simulink model "myo_sfun_one_myo_imu_emg"  (R2019a)
(part 5 of 12)

  "IW{2,1}(261,:)'" : Constant  Value=[-0.5347940637473553859848607316962443292140960693359375;-0.259539238988193254886738259301637299358844757080078125;-0.7408074576731140670204922571429051458835601806640625;-0.40336307327878595518910742612206377089023590087890625;-1.55843068978388021861292145331390202045440673828125;1.7382673124555321209072644705884158611297607421875;1.5250036038475383026735698877018876373767852783203125;1.420255341369331514300711205578409135341644287109375]
      mask Display: e = 0.06;c1 = [120 150 230]/255;c2 = ([120 150 230]+0)/383;c3 = ([120 150 230]+128)/383;patch([0 1 1 0],[0 0 1 1],c1);patch([0 1 1 1-e 1-e 0+e],[0 0 1 1-e 0+e 0+e],c2);patch([0 0 1 1-e 0+e 0+e],[0 1 1 1-e 1-e 0+e],c3);plot([0 1 1 0 0],[0 0 1 1 0]);disp('weights');
  "IW{2,1}(262,:)'" : Constant  Value=[-1.2137447248221431284065374711644835770130157470703125;1.3683347708584874258264107993454672396183013916015625;1.5705948868795653883267959827207960188388824462890625;0.11601457680919935455676750279963016510009765625;0.762641288467723388322383470949716866016387939453125;0.40056359138445618572887951813754625618457794189453125;0.9697544812676659464756312445388175547122955322265625;-1.8867637485871338043352807289920747280120849609375]
      mask Display: e = 0.06;c1 = [120 150 230]/255;c2 = ([120 150 230]+0)/383;c3 = ([120 150 230]+128)/383;patch([0 1 1 0],[0 0 1 1],c1);patch([0 1 1 1-e 1-e 0+e],[0 0 1 1-e 0+e 0+e],c2);patch([0 0 1 1-e 0+e 0+e],[0 1 1 1-e 1-e 0+e],c3);plot([0 1 1 0 0],[0 0 1 1 0]);disp('weights');
  "IW{2,1}(263,:)'" : Constant  Value=[0.96222248705589408235283599424292333424091339111328125;-1.7544566772263916476504164165817201137542724609375;-0.7898635199195138678618377525708638131618499755859375;1.1345806161849127935425940449931658804416656494140625;1.2407133822809399692488341315765865147113800048828125;1.6768418735501995353587290082941763103008270263671875;0.8817648711825756269178100410499610006809234619140625;-0.3888922972442336867260337385232560336589813232421875]
      mask Display: e = 0.06;c1 = [120 150 230]/255;c2 = ([120 150 230]+0)/383;c3 = ([120 150 230]+128)/383;patch([0 1 1 0],[0 0 1 1],c1);patch([0 1 1 1-e 1-e 0+e],[0 0 1 1-e 0+e 0+e],c2);patch([0 0 1 1-e 0+e 0+e],[0 1 1 1-e 1-e 0+e],c3);plot([0 1 1 0 0],[0 0 1 1 0]);disp('weights');
  "IW{2,1}(264,:)'" : Constant  Value=[-1.5476465341889766857974564118194393813610076904296875;1.326692801950664080123942767386324703693389892578125;-1.4681341462454096102874245843850076198577880859375;-0.46925473122198557707207555722561664879322052001953125;1.2734078675367908051185850126785226166248321533203125;0.56485698316167909371898758763563819229602813720703125;-0.88411430126475953894527037846273742616176605224609375;1.345718049246266811991290524019859731197357177734375]
      mask Display: e = 0.06;c1 = [120 150 230]/255;c2 = ([120 150 230]+0)/383;c3 = ([120 150 230]+128)/383;patch([0 1 1 0],[0 0 1 1],c1);patch([0 1 1 1-e 1-e 0+e],[0 0 1 1-e 0+e 0+e],c2);patch([0 0 1 1-e 0+e 0+e],[0 1 1 1-e 1-e 0+e],c3);plot([0 1 1 0 0],[0 0 1 1 0]);disp('weights');
  "IW{2,1}(265,:)'" : Constant  Value=[1.3669130157252069590612109095673076808452606201171875;0.38000314021766767869081604658276773989200592041015625;1.4510424437195197366889942713896743953227996826171875;1.132229379854207795830234317691065371036529541015625;-0.7653685535385428284627096218173392117023468017578125;-1.6459644702436435625969579632510431110858917236328125;-1.210523284810293365154620914836414158344268798828125;-0.87108616897754220786964651779271662235260009765625]
      mask Display: e = 0.06;c1 = [120 150 230]/255;c2 = ([120 150 230]+0)/383;c3 = ([120 150 230]+128)/383;patch([0 1 1 0],[0 0 1 1],c1);patch([0 1 1 1-e 1-e 0+e],[0 0 1 1-e 0+e 0+e],c2);patch([0 0 1 1-e 0+e 0+e],[0 1 1 1-e 1-e 0+e],c3);plot([0 1 1 0 0],[0 0 1 1 0]);disp('weights');
  "IW{2,1}(266,:)'" : Constant  Value=[1.5789125748257089032478006629389710724353790283203125;-1.7464317776296429673976717822370119392871856689453125;0.989813563582735422841096806223504245281219482421875;0.93718327672771994940603690338321030139923095703125;-1.0300358206486419643255203482112847268581390380859375;-0.33243528081857032230317372523131780326366424560546875;-0.048545225170301485595469870304441428743302822113037109375;1.6203864687595086468974159288336522877216339111328125]
      mask Display: e = 0.06;c1 = [120 150 230]/255;c2 = ([120 150 230]+0)/383;c3 = ([120 150 230]+128)/383;patch([0 1 1 0],[0 0 1 1],c1);patch([0 1 1 1-e 1-e 0+e],[0 0 1 1-e 0+e 0+e],c2);patch([0 0 1 1-e 0+e 0+e],[0 1 1 1-e 1-e 0+e],c3);plot([0 1 1 0 0],[0 0 1 1 0]);disp('weights');
  "IW{2,1}(267,:)'" : Constant  Value=[-1.88334330389469162270188462571240961551666259765625;-1.550976382192118752101350764860399067401885986328125;1.4240772823814003000819639055407606065273284912109375;0.82226012569760731363288641659892164170742034912109375;-0.78530498389310732232360123816761188209056854248046875;-0.9885174017696252146691904272302053868770599365234375;0.9423763715994548650911610820912756025791168212890625;-0.4230164293665026331581202612142078578472137451171875]
      mask Display: e = 0.06;c1 = [120 150 230]/255;c2 = ([120 150 230]+0)/383;c3 = ([120 150 230]+128)/383;patch([0 1 1 0],[0 0 1 1],c1);patch([0 1 1 1-e 1-e 0+e],[0 0 1 1-e 0+e 0+e],c2);patch([0 0 1 1-e 0+e 0+e],[0 1 1 1-e 1-e 0+e],c3);plot([0 1 1 0 0],[0 0 1 1 0]);disp('weights');
  "IW{2,1}(268,:)'" : Constant  Value=[0.77703759880490519407203464652411639690399169921875;0.431370173463836492633305397248477675020694732666015625;-1.1019623341089503920642300727195106446743011474609375;1.719390729815739593533407969516701996326446533203125;0.70250763369316004958164967320044524967670440673828125;-1.8212153285883927456012543188990093767642974853515625;0.078282166399910979581733272425481118261814117431640625;1.5732714658743549573927111850935034453868865966796875]
      mask Display: e = 0.06;c1 = [120 150 230]/255;c2 = ([120 150 230]+0)/383;c3 = ([120 150 230]+128)/383;patch([0 1 1 0],[0 0 1 1],c1);patch([0 1 1 1-e 1-e 0+e],[0 0 1 1-e 0+e 0+e],c2);patch([0 0 1 1-e 0+e 0+e],[0 1 1 1-e 1-e 0+e],c3);plot([0 1 1 0 0],[0 0 1 1 0]);disp('weights');
  "IW{2,1}(269,:)'" : Constant  Value=[0.358805185099290657735338072598096914589405059814453125;-0.85788688273212521107069505887920968234539031982421875;0.6189663674455470054880379393580369651317596435546875;0.3732430252180132246309085530810989439487457275390625;-1.52643420461756118555740613373927772045135498046875;-0.8164779329250595463207673674332909286022186279296875;-1.966212472493690910368968616239726543426513671875;1.6658060255045030739751155124395154416561126708984375]
      mask Display: e = 0.06;c1 = [120 150 230]/255;c2 = ([120 150 230]+0)/383;c3 = ([120 150 230]+128)/383;patch([0 1 1 0],[0 0 1 1],c1);patch([0 1 1 1-e 1-e 0+e],[0 0 1 1-e 0+e 0+e],c2);patch([0 0 1 1-e 0+e 0+e],[0 1 1 1-e 1-e 0+e],c3);plot([0 1 1 0 0],[0 0 1 1 0]);disp('weights');
  "IW{2,1}(27,:)'" : Constant  Value=[1.0976471878022999728585773482336662709712982177734375;-1.466978524772944769694049682584591209888458251953125;-0.06567386280703979561934602315886877477169036865234375;-0.90721269995288233989327864037477411329746246337890625;-0.5755879150808522748405948732397519052028656005859375;-1.2134225702139129765555480844341218471527099609375;1.689553489070515723824428278021514415740966796875;-1.478611033845023126076512198778800666332244873046875]
      mask Display: e = 0.06;c1 = [120 150 230]/255;c2 = ([120 150 230]+0)/383;c3 = ([120 150 230]+128)/383;patch([0 1 1 0],[0 0 1 1],c1);patch([0 1 1 1-e 1-e 0+e],[0 0 1 1-e 0+e 0+e],c2);patch([0 0 1 1-e 0+e 0+e],[0 1 1 1-e 1-e 0+e],c3);plot([0 1 1 0 0],[0 0 1 1 0]);disp('weights');
  "IW{2,1}(270,:)'" : Constant  Value=[1.4595164985252182532349252142012119293212890625;-0.359501600059089099215015039590070955455303192138671875;0.096861650405547894404634234888362698256969451904296875;-1.49178391212668426391019238508306443691253662109375;1.389601437905864766975128077319823205471038818359375;0.373202055967952806003751220487174578011035919189453125;1.851491441376186042333529258030466735363006591796875;-1.073163490086033622361583184101618826389312744140625]
      mask Display: e = 0.06;c1 = [120 150 230]/255;c2 = ([120 150 230]+0)/383;c3 = ([120 150 230]+128)/383;patch([0 1 1 0],[0 0 1 1],c1);patch([0 1 1 1-e 1-e 0+e],[0 0 1 1-e 0+e 0+e],c2);patch([0 0 1 1-e 0+e 0+e],[0 1 1 1-e 1-e 0+e],c3);plot([0 1 1 0 0],[0 0 1 1 0]);disp('weights');
  "IW{2,1}(271,:)'" : Constant  Value=[0.97058856146866234748671331544755958020687103271484375;-0.65670569787586685617242210355470888316631317138671875;-0.5609898191570097392144589321105740964412689208984375;-0.9346593350875387340437328020925633609294891357421875;-0.9836655602936890119281088118441402912139892578125;2.248750882651939786427419676329009234905242919921875;-1.32453501057655298467352622537873685359954833984375;0.86687601885010667768227676788228563964366912841796875]
      mask Display: e = 0.06;c1 = [120 150 230]/255;c2 = ([120 150 230]+0)/383;c3 = ([120 150 230]+128)/383;patch([0 1 1 0],[0 0 1 1],c1);patch([0 1 1 1-e 1-e 0+e],[0 0 1 1-e 0+e 0+e],c2);patch([0 0 1 1-e 0+e 0+e],[0 1 1 1-e 1-e 0+e],c3);plot([0 1 1 0 0],[0 0 1 1 0]);disp('weights');
  "IW{2,1}(272,:)'" : Constant  Value=[-1.32787760878514671247785372543148696422576904296875;0.84357176605215411502314282188308425247669219970703125;0.455621916527780113082002344526699744164943695068359375;-0.7202920248291266869244964254903607070446014404296875;1.0883011856233171243957258411683142185211181640625;-1.6432271653339125538906273504835553467273712158203125;0.82982796555327198451124104394693858921527862548828125;1.7873354043180602612750362823135219514369964599609375]
      mask Display: e = 0.06;c1 = [120 150 230]/255;c2 = ([120 150 230]+0)/383;c3 = ([120 150 230]+128)/383;patch([0 1 1 0],[0 0 1 1],c1);patch([0 1 1 1-e 1-e 0+e],[0 0 1 1-e 0+e 0+e],c2);patch([0 0 1 1-e 0+e 0+e],[0 1 1 1-e 1-e 0+e],c3);plot([0 1 1 0 0],[0 0 1 1 0]);disp('weights');
  "IW{2,1}(273,:)'" : Constant  Value=[-1.43578424813973182239124071202240884304046630859375;-1.8517703535549074889132725729723460972309112548828125;0.41544081412662092755994081016979180276393890380859375;-1.091247752457320530083961784839630126953125;-0.196299549298969033817030549471382983028888702392578125;-0.95868845801884028379191704516415484249591827392578125;1.2310815496712879113516692086705006659030914306640625;-1.3264965863304400972566554628429003059864044189453125]
      mask Display: e = 0.06;c1 = [120 150 230]/255;c2 = ([120 150 230]+0)/383;c3 = ([120 150 230]+128)/383;patch([0 1 1 0],[0 0 1 1],c1);patch([0 1 1 1-e 1-e 0+e],[0 0 1 1-e 0+e 0+e],c2);patch([0 0 1 1-e 0+e 0+e],[0 1 1 1-e 1-e 0+e],c3);plot([0 1 1 0 0],[0 0 1 1 0]);disp('weights');
  "IW{2,1}(274,:)'" : Constant  Value=[-0.95662628683772410465024904624442569911479949951171875;-1.0981679705156925930253919432288967072963714599609375;1.5430734491925364171294177140225656330585479736328125;-0.1038975800053978659764908343277056701481342315673828125;1.3390766380696075277256795743596740067005157470703125;0.9747187685846545601719981277710758149623870849609375;-0.63364061371546254175513013251475058495998382568359375;1.841906858781021671944699846790172159671783447265625]
      mask Display: e = 0.06;c1 = [120 150 230]/255;c2 = ([120 150 230]+0)/383;c3 = ([120 150 230]+128)/383;patch([0 1 1 0],[0 0 1 1],c1);patch([0 1 1 1-e 1-e 0+e],[0 0 1 1-e 0+e 0+e],c2);patch([0 0 1 1-e 0+e 0+e],[0 1 1 1-e 1-e 0+e],c3);plot([0 1 1 0 0],[0 0 1 1 0]);disp('weights');
  "IW{2,1}(275,:)'" : Constant  Value=[-0.34169892612024443945273333156364969909191131591796875;-0.89637397571807053697767742050928063690662384033203125;1.1176334887777461535307566009578295052051544189453125;2.103754722856508774242456638603471219539642333984375;1.3408946331418707398341894077020697295665740966796875;-1.33424973593796547532974727801047265529632568359375;0.59089858131655770279166972613893449306488037109375;-0.7138255704883051944165117674856446683406829833984375]
      mask Display: e = 0.06;c1 = [120 150 230]/255;c2 = ([120 150 230]+0)/383;c3 = ([120 150 230]+128)/383;patch([0 1 1 0],[0 0 1 1],c1);patch([0 1 1 1-e 1-e 0+e],[0 0 1 1-e 0+e 0+e],c2);patch([0 0 1 1-e 0+e 0+e],[0 1 1 1-e 1-e 0+e],c3);plot([0 1 1 0 0],[0 0 1 1 0]);disp('weights');
  "IW{2,1}(276,:)'" : Constant  Value=[-1.3416184792027767702649043712881393730640411376953125;1.4813472558584823701721688848920166492462158203125;1.449577220120267018188542351708747446537017822265625;1.97812474261925874685630333260633051395416259765625;0.161596659980792811683869558692094869911670684814453125;-0.644855468938165810044438330805860459804534912109375;0.511488114681550865014969531330280005931854248046875;0.54368784143616533111043054304900579154491424560546875]
      mask Display: e = 0.06;c1 = [120 150 230]/255;c2 = ([120 150 230]+0)/383;c3 = ([120 150 230]+128)/383;patch([0 1 1 0],[0 0 1 1],c1);patch([0 1 1 1-e 1-e 0+e],[0 0 1 1-e 0+e 0+e],c2);patch([0 0 1 1-e 0+e 0+e],[0 1 1 1-e 1-e 0+e],c3);plot([0 1 1 0 0],[0 0 1 1 0]);disp('weights');
  "IW{2,1}(277,:)'" : Constant  Value=[-1.735736727684186408993127770372666418552398681640625;1.4868573855134827876867120721726678311824798583984375;-1.5646534212947937891868832593900151550769805908203125;0.400031089853374488551907006694818846881389617919921875;-0.024142580804420908646701349198337993584573268890380859375;0.780105394974893950887917526415549218654632568359375;0.85181123327748242690660163134452886879444122314453125;1.3627409629516336053711711429059505462646484375]
      mask Display: e = 0.06;c1 = [120 150 230]/255;c2 = ([120 150 230]+0)/383;c3 = ([120 150 230]+128)/383;patch([0 1 1 0],[0 0 1 1],c1);patch([0 1 1 1-e 1-e 0+e],[0 0 1 1-e 0+e 0+e],c2);patch([0 0 1 1-e 0+e 0+e],[0 1 1 1-e 1-e 0+e],c3);plot([0 1 1 0 0],[0 0 1 1 0]);disp('weights');
  "IW{2,1}(278,:)'" : Constant  Value=[-1.56186260805010501684364498942159116268157958984375;-1.100006899394458059759926982223987579345703125;1.560648778966891025987706598243676126003265380859375;1.4873168322882188707723116749548353254795074462890625;0.46043106493486385399904747828259132802486419677734375;0.185967771515183122321701603141264058649539947509765625;1.4417075965386454416972128456109203398227691650390625;-0.53803330954568850952313141533522866666316986083984375]
      mask Display: e = 0.06;c1 = [120 150 230]/255;c2 = ([120 150 230]+0)/383;c3 = ([120 150 230]+128)/383;patch([0 1 1 0],[0 0 1 1],c1);patch([0 1 1 1-e 1-e 0+e],[0 0 1 1-e 0+e 0+e],c2);patch([0 0 1 1-e 0+e 0+e],[0 1 1 1-e 1-e 0+e],c3);plot([0 1 1 0 0],[0 0 1 1 0]);disp('weights');
  "IW{2,1}(279,:)'" : Constant  Value=[-0.36281345583298441059838523869984783232212066650390625;1.4390043629114261936052798773744143545627593994140625;0.06453072679456033078349008746954496018588542938232421875;1.05104162461502159686688173678703606128692626953125;-1.5431302947782772339024859320488758385181427001953125;-0.93221088137758789660125557929859496653079986572265625;0.267812486808182315112247806609957478940486907958984375;2.097864843359056319371802601381205022335052490234375]
      mask Display: e = 0.06;c1 = [120 150 230]/255;c2 = ([120 150 230]+0)/383;c3 = ([120 150 230]+128)/383;patch([0 1 1 0],[0 0 1 1],c1);patch([0 1 1 1-e 1-e 0+e],[0 0 1 1-e 0+e 0+e],c2);patch([0 0 1 1-e 0+e 0+e],[0 1 1 1-e 1-e 0+e],c3);plot([0 1 1 0 0],[0 0 1 1 0]);disp('weights');
  "IW{2,1}(28,:)'" : Constant  Value=[-0.90251119652570188645057669418747536838054656982421875;1.9962297316221044862771805128431878983974456787109375;2.10309210297034088199552570586092770099639892578125;-1.0280337214971939641117160135763697326183319091796875;0.519169850362849683023114266688935458660125732421875;0.58015023794351805452862436141003854572772979736328125;0.1759229481877064016348555242075235582888126373291015625;0.326899828584390539365500671920017339289188385009765625]
      mask Display: e = 0.06;c1 = [120 150 230]/255;c2 = ([120 150 230]+0)/383;c3 = ([120 150 230]+128)/383;patch([0 1 1 0],[0 0 1 1],c1);patch([0 1 1 1-e 1-e 0+e],[0 0 1 1-e 0+e 0+e],c2);patch([0 0 1 1-e 0+e 0+e],[0 1 1 1-e 1-e 0+e],c3);plot([0 1 1 0 0],[0 0 1 1 0]);disp('weights');
  "IW{2,1}(280,:)'" : Constant  Value=[1.126874992238202199956731419661082327365875244140625;-0.310662957071799805675027528195641934871673583984375;1.3794381468792427103409181654569692909717559814453125;-1.1011192837083199069780903300852514803409576416015625;1.2389242018177260007405493524856865406036376953125;0.2294867389644391353353825024896650575101375579833984375;1.0441557628103759203241907016490586102008819580078125;1.9669664675496492112216628811438567936420440673828125]
      mask Display: e = 0.06;c1 = [120 150 230]/255;c2 = ([120 150 230]+0)/383;c3 = ([120 150 230]+128)/383;patch([0 1 1 0],[0 0 1 1],c1);patch([0 1 1 1-e 1-e 0+e],[0 0 1 1-e 0+e 0+e],c2);patch([0 0 1 1-e 0+e 0+e],[0 1 1 1-e 1-e 0+e],c3);plot([0 1 1 0 0],[0 0 1 1 0]);disp('weights');
  "IW{2,1}(281,:)'" : Constant  Value=[0.483592536764545333216602784887072630226612091064453125;-2.158889894419294019911603754735551774501800537109375;-1.05987617340272688437607939704321324825286865234375;0.69486367072161192570689536296413280069828033447265625;1.1198683344627422542316708131693303585052490234375;-1.1965790950295855932239419416873715817928314208984375;-0.9931210388714486470007614116184413433074951171875;-0.942888086306401529412823947495780885219573974609375]
      mask Display: e = 0.06;c1 = [120 150 230]/255;c2 = ([120 150 230]+0)/383;c3 = ([120 150 230]+128)/383;patch([0 1 1 0],[0 0 1 1],c1);patch([0 1 1 1-e 1-e 0+e],[0 0 1 1-e 0+e 0+e],c2);patch([0 0 1 1-e 0+e 0+e],[0 1 1 1-e 1-e 0+e],c3);plot([0 1 1 0 0],[0 0 1 1 0]);disp('weights');
  "IW{2,1}(282,:)'" : Constant  Value=[0.91468655581167979118362154622445814311504364013671875;-1.1775706258562699257907979699666611850261688232421875;-0.96927585702251750632285620667971670627593994140625;-1.3837978877602832294968493442866019904613494873046875;1.3407367494679702790705277948291040956974029541015625;1.075182371223083688249744227505289018154144287109375;-1.410665767931468916884796271915547549724578857421875;1.0674170493635213308181164393317885696887969970703125]
      mask Display: e = 0.06;c1 = [120 150 230]/255;c2 = ([120 150 230]+0)/383;c3 = ([120 150 230]+128)/383;patch([0 1 1 0],[0 0 1 1],c1);patch([0 1 1 1-e 1-e 0+e],[0 0 1 1-e 0+e 0+e],c2);patch([0 0 1 1-e 0+e 0+e],[0 1 1 1-e 1-e 0+e],c3);plot([0 1 1 0 0],[0 0 1 1 0]);disp('weights');
  "IW{2,1}(283,:)'" : Constant  Value=[-1.3783752363382208994124766832101158797740936279296875;1.0054603651816405029961742911837063729763031005859375;-1.494867039260532326494512744829989969730377197265625;1.0665452392347567478481096259201876819133758544921875;1.018899772728071528860027683549560606479644775390625;-1.285845475365987145011104075820185244083404541015625;-1.429423307222606798205788436462171375751495361328125;-0.10322951687595514902451299121821648441255092620849609375]
      mask Display: e = 0.06;c1 = [120 150 230]/255;c2 = ([120 150 230]+0)/383;c3 = ([120 150 230]+128)/383;patch([0 1 1 0],[0 0 1 1],c1);patch([0 1 1 1-e 1-e 0+e],[0 0 1 1-e 0+e 0+e],c2);patch([0 0 1 1-e 0+e 0+e],[0 1 1 1-e 1-e 0+e],c3);plot([0 1 1 0 0],[0 0 1 1 0]);disp('weights');
  "IW{2,1}(284,:)'" : Constant  Value=[0.1572972901949951374245273427732172422111034393310546875;-1.2723462678150279092648133882903493940830230712890625;1.561837886277977371918268545414321124553680419921875;1.741138590659697005236239419900812208652496337890625;0.83441033896946625869617264470434747636318206787109375;-0.039011284281160678311106693172405357472598552703857421875;1.7881067609712910648767092425259761512279510498046875;-0.2145482555579586725347240871997200883924961090087890625]
      mask Display: e = 0.06;c1 = [120 150 230]/255;c2 = ([120 150 230]+0)/383;c3 = ([120 150 230]+128)/383;patch([0 1 1 0],[0 0 1 1],c1);patch([0 1 1 1-e 1-e 0+e],[0 0 1 1-e 0+e 0+e],c2);patch([0 0 1 1-e 0+e 0+e],[0 1 1 1-e 1-e 0+e],c3);plot([0 1 1 0 0],[0 0 1 1 0]);disp('weights');
  "IW{2,1}(285,:)'" : Constant  Value=[-1.116838898596282714237304389826022088527679443359375;-0.45361005852011071493024019218864850699901580810546875;-0.1467195540551750887470205952922697179019451141357421875;-0.77123417068573274502085723725031130015850067138671875;-1.01269951209783659606955552590079605579376220703125;-1.536443689826322067659702952369116246700286865234375;0.7644814837354527714552432371419854462146759033203125;2.219712582372310283318483925540931522846221923828125]
      mask Display: e = 0.06;c1 = [120 150 230]/255;c2 = ([120 150 230]+0)/383;c3 = ([120 150 230]+128)/383;patch([0 1 1 0],[0 0 1 1],c1);patch([0 1 1 1-e 1-e 0+e],[0 0 1 1-e 0+e 0+e],c2);patch([0 0 1 1-e 0+e 0+e],[0 1 1 1-e 1-e 0+e],c3);plot([0 1 1 0 0],[0 0 1 1 0]);disp('weights');
  "IW{2,1}(286,:)'" : Constant  Value=[0.1995306126975101845832938352032215334475040435791015625;-1.7161681488379654236808846690109930932521820068359375;-1.480581408540153187658461320097558200359344482421875;-1.537504376924896387635044447961263358592987060546875;-1.7887266527028222729001072366372682154178619384765625;-0.1609063893290709479355626854157890193164348602294921875;0.05322388997146536293580965093497070483863353729248046875;-0.50484691917346913303532573991105891764163970947265625]
      mask Display: e = 0.06;c1 = [120 150 230]/255;c2 = ([120 150 230]+0)/383;c3 = ([120 150 230]+128)/383;patch([0 1 1 0],[0 0 1 1],c1);patch([0 1 1 1-e 1-e 0+e],[0 0 1 1-e 0+e 0+e],c2);patch([0 0 1 1-e 0+e 0+e],[0 1 1 1-e 1-e 0+e],c3);plot([0 1 1 0 0],[0 0 1 1 0]);disp('weights');
  "IW{2,1}(287,:)'" : Constant  Value=[-0.94112595153402944792020434761070646345615386962890625;-0.99001731697002182119859980957699008285999298095703125;1.8620901433696148696839145486592315137386322021484375;-0.6551074243207744007833071009372361004352569580078125;-0.1610648165904539907966608325295965187251567840576171875;0.89392555591680811222232705404167063534259796142578125;-2.086354445914893052105298920650966465473175048828125;-0.1826483784180093772331332502290024422109127044677734375]
      mask Display: e = 0.06;c1 = [120 150 230]/255;c2 = ([120 150 230]+0)/383;c3 = ([120 150 230]+128)/383;patch([0 1 1 0],[0 0 1 1],c1);patch([0 1 1 1-e 1-e 0+e],[0 0 1 1-e 0+e 0+e],c2);patch([0 0 1 1-e 0+e 0+e],[0 1 1 1-e 1-e 0+e],c3);plot([0 1 1 0 0],[0 0 1 1 0]);disp('weights');
  "IW{2,1}(288,:)'" : Constant  Value=[0.52458174714693217577377026827889494597911834716796875;1.7398230354122528051874496668460778892040252685546875;-1.519901214688633928062699851579964160919189453125;-0.86917209525089400568020892023923806846141815185546875;0.92940725891443654038681643214658834040164947509765625;1.2385217255743719011462644630228169262409210205078125;-1.58607583101517501944499599630944430828094482421875;-0.1160806490231749144026451858735526911914348602294921875]
      mask Display: e = 0.06;c1 = [120 150 230]/255;c2 = ([120 150 230]+0)/383;c3 = ([120 150 230]+128)/383;patch([0 1 1 0],[0 0 1 1],c1);patch([0 1 1 1-e 1-e 0+e],[0 0 1 1-e 0+e 0+e],c2);patch([0 0 1 1-e 0+e 0+e],[0 1 1 1-e 1-e 0+e],c3);plot([0 1 1 0 0],[0 0 1 1 0]);disp('weights');
  "IW{2,1}(289,:)'" : Constant  Value=[-1.2917048065390790423379030471551232039928436279296875;-0.71049630680784592318133263688650913536548614501953125;0.86402303793719081870250420251977629959583282470703125;-1.1367972813391349351519465926685370504856109619140625;1.765463373969804905527780647389590740203857421875;-0.39553717415411515645473627955652773380279541015625;-1.3503491957773159359845749349915422499179840087890625;1.303257147695879414328601342276670038700103759765625]
      mask Display: e = 0.06;c1 = [120 150 230]/255;c2 = ([120 150 230]+0)/383;c3 = ([120 150 230]+128)/383;patch([0 1 1 0],[0 0 1 1],c1);patch([0 1 1 1-e 1-e 0+e],[0 0 1 1-e 0+e 0+e],c2);patch([0 0 1 1-e 0+e 0+e],[0 1 1 1-e 1-e 0+e],c3);plot([0 1 1 0 0],[0 0 1 1 0]);disp('weights');
  "IW{2,1}(29,:)'" : Constant  Value=[-1.7090129519907464317185485924710519611835479736328125;-1.3034815042726444200837931930436752736568450927734375;-1.351266315762916558895767593639902770519256591796875;0.67773782565702356261994054875685833394527435302734375;0.78014348610426365038250651195994578301906585693359375;-0.62637339626419696880788023918285034596920013427734375;-1.20017218462587482719072795589454472064971923828125;1.4139008249440487841042113359435461461544036865234375]
      mask Display: e = 0.06;c1 = [120 150 230]/255;c2 = ([120 150 230]+0)/383;c3 = ([120 150 230]+128)/383;patch([0 1 1 0],[0 0 1 1],c1);patch([0 1 1 1-e 1-e 0+e],[0 0 1 1-e 0+e 0+e],c2);patch([0 0 1 1-e 0+e 0+e],[0 1 1 1-e 1-e 0+e],c3);plot([0 1 1 0 0],[0 0 1 1 0]);disp('weights');
  "IW{2,1}(290,:)'" : Constant  Value=[0.56386891610408518271668754096026532351970672607421875;-0.08552175739171119506210061445017345249652862548828125;1.1462792767544254246558921295218169689178466796875;-1.68939509070532078993664981680922210216522216796875;1.6352454019301372323269561093184165656566619873046875;1.517885155302728161785807969863526523113250732421875;-0.56379379957213171525864936484140343964099884033203125;1.0920500642273209823684965158463455736637115478515625]
      mask Display: e = 0.06;c1 = [120 150 230]/255;c2 = ([120 150 230]+0)/383;c3 = ([120 150 230]+128)/383;patch([0 1 1 0],[0 0 1 1],c1);patch([0 1 1 1-e 1-e 0+e],[0 0 1 1-e 0+e 0+e],c2);patch([0 0 1 1-e 0+e 0+e],[0 1 1 1-e 1-e 0+e],c3);plot([0 1 1 0 0],[0 0 1 1 0]);disp('weights');
  "IW{2,1}(291,:)'" : Constant  Value=[1.23373218350272306764736640616320073604583740234375;-1.3373685199427944869654538706527091562747955322265625;0.48442904663986230406891309030470438301563262939453125;-0.1576922269796413866860262942282133735716342926025390625;0.417134833136712346313146326792775653302669525146484375;0.74684790145846158271325521127437241375446319580078125;-1.515155489828451162992450917954556643962860107421875;2.1078436254838255337062946637161076068878173828125]
      mask Display: e = 0.06;c1 = [120 150 230]/255;c2 = ([120 150 230]+0)/383;c3 = ([120 150 230]+128)/383;patch([0 1 1 0],[0 0 1 1],c1);patch([0 1 1 1-e 1-e 0+e],[0 0 1 1-e 0+e 0+e],c2);patch([0 0 1 1-e 0+e 0+e],[0 1 1 1-e 1-e 0+e],c3);plot([0 1 1 0 0],[0 0 1 1 0]);disp('weights');
  "IW{2,1}(292,:)'" : Constant  Value=[0.149355769972121577016110904878587462007999420166015625;-1.797772213812643737895768936141394078731536865234375;1.7712538370147437039037185968481935560703277587890625;-1.0021657351335420127469433282385580241680145263671875;0.1743328572903561635154545683690230362117290496826171875;-1.4389073129166494169339785003103315830230712890625;-0.87641589879673664764681007000035606324672698974609375;0.8661315996802823047318042881670407950878143310546875]
      mask Display: e = 0.06;c1 = [120 150 230]/255;c2 = ([120 150 230]+0)/383;c3 = ([120 150 230]+128)/383;patch([0 1 1 0],[0 0 1 1],c1);patch([0 1 1 1-e 1-e 0+e],[0 0 1 1-e 0+e 0+e],c2);patch([0 0 1 1-e 0+e 0+e],[0 1 1 1-e 1-e 0+e],c3);plot([0 1 1 0 0],[0 0 1 1 0]);disp('weights');
  "IW{2,1}(293,:)'" : Constant  Value=[0.15491241101211217223720950642018578946590423583984375;0.16704681014463995669672158328467048704624176025390625;-1.0391931780589243050627601405722089111804962158203125;-2.043870802913976714165755765861831605434417724609375;-1.8472817074879319676483646617271006107330322265625;1.2477502395181587768746567235211841762065887451171875;-0.88279567899519839624389305754448287189006805419921875;0.03624299588909961344906918156993924640119075775146484375]
      mask Display: e = 0.06;c1 = [120 150 230]/255;c2 = ([120 150 230]+0)/383;c3 = ([120 150 230]+128)/383;patch([0 1 1 0],[0 0 1 1],c1);patch([0 1 1 1-e 1-e 0+e],[0 0 1 1-e 0+e 0+e],c2);patch([0 0 1 1-e 0+e 0+e],[0 1 1 1-e 1-e 0+e],c3);plot([0 1 1 0 0],[0 0 1 1 0]);disp('weights');
  "IW{2,1}(294,:)'" : Constant  Value=[-1.5072503309985483266331129925674758851528167724609375;-0.5912296405544983368685052482760511338710784912109375;-1.8839554420834103698467743015498854219913482666015625;-0.211657758410721930086850761654204688966274261474609375;-0.287930466127750139815333341175573877990245819091796875;0.281307788952104342872218012416851706802845001220703125;-1.9679232919960212289112178041250444948673248291015625;-0.80560222171074702401938338880427181720733642578125]
      mask Display: e = 0.06;c1 = [120 150 230]/255;c2 = ([120 150 230]+0)/383;c3 = ([120 150 230]+128)/383;patch([0 1 1 0],[0 0 1 1],c1);patch([0 1 1 1-e 1-e 0+e],[0 0 1 1-e 0+e 0+e],c2);patch([0 0 1 1-e 0+e 0+e],[0 1 1 1-e 1-e 0+e],c3);plot([0 1 1 0 0],[0 0 1 1 0]);disp('weights');
  "IW{2,1}(295,:)'" : Constant  Value=[0.12344705431950199481239138776800245977938175201416015625;-1.6339196595745466566995673929341137409210205078125;1.674123558913491738309176071197725832462310791015625;1.6729989118184416252432811234029941260814666748046875;0.54506681304176629598856607117340900003910064697265625;0.708510405456726832795766313211061060428619384765625;1.3533935295393735298574711123364977538585662841796875;-0.26785656899876630898660323509830050170421600341796875]
      mask Display: e = 0.06;c1 = [120 150 230]/255;c2 = ([120 150 230]+0)/383;c3 = ([120 150 230]+128)/383;patch([0 1 1 0],[0 0 1 1],c1);patch([0 1 1 1-e 1-e 0+e],[0 0 1 1-e 0+e 0+e],c2);patch([0 0 1 1-e 0+e 0+e],[0 1 1 1-e 1-e 0+e],c3);plot([0 1 1 0 0],[0 0 1 1 0]);disp('weights');
  "IW{2,1}(296,:)'" : Constant  Value=[-1.3048676985666547434306039576767943799495697021484375;1.643205394783701311922641252749599516391754150390625;0.1963040358895786763326896107173524796962738037109375;-1.244179839042650836944403636152856051921844482421875;0.930456184365194172158908259007148444652557373046875;-0.3428724376575236210129560276982374489307403564453125;-1.9619371156705327496894142313976772129535675048828125;-0.7667766256128121238333505971240811049938201904296875]
      mask Display: e = 0.06;c1 = [120 150 230]/255;c2 = ([120 150 230]+0)/383;c3 = ([120 150 230]+128)/383;patch([0 1 1 0],[0 0 1 1],c1);patch([0 1 1 1-e 1-e 0+e],[0 0 1 1-e 0+e 0+e],c2);patch([0 0 1 1-e 0+e 0+e],[0 1 1 1-e 1-e 0+e],c3);plot([0 1 1 0 0],[0 0 1 1 0]);disp('weights');
  "IW{2,1}(297,:)'" : Constant  Value=[0.7318966623372527013913213522755540907382965087890625;0.98989772384461360843488364480435848236083984375;-1.4657202518633074550535866364953108131885528564453125;-0.67854688032233922978520013202796690165996551513671875;-0.739015982277783312071051113889552652835845947265625;-1.4522550716225806066717041176161728799343109130859375;1.6168939132434669847526720332098193466663360595703125;-1.2758844453122988316096098060370422899723052978515625]
      mask Display: e = 0.06;c1 = [120 150 230]/255;c2 = ([120 150 230]+0)/383;c3 = ([120 150 230]+128)/383;patch([0 1 1 0],[0 0 1 1],c1);patch([0 1 1 1-e 1-e 0+e],[0 0 1 1-e 0+e 0+e],c2);patch([0 0 1 1-e 0+e 0+e],[0 1 1 1-e 1-e 0+e],c3);plot([0 1 1 0 0],[0 0 1 1 0]);disp('weights');
  "IW{2,1}(298,:)'" : Constant  Value=[1.209392504203771867565819775336422026157379150390625;1.2760262193505449435093623833381570875644683837890625;-0.66825151936986804113161042550927959382534027099609375;-1.694680276642486216331917603383772075176239013671875;-0.99422304321615195821237875861697830259799957275390625;-0.03750831860010338247857220039804815314710140228271484375;-1.392430533587185603749958318076096475124359130859375;-1.2927934329263728319148185619269497692584991455078125]
      mask Display: e = 0.06;c1 = [120 150 230]/255;c2 = ([120 150 230]+0)/383;c3 = ([120 150 230]+128)/383;patch([0 1 1 0],[0 0 1 1],c1);patch([0 1 1 1-e 1-e 0+e],[0 0 1 1-e 0+e 0+e],c2);patch([0 0 1 1-e 0+e 0+e],[0 1 1 1-e 1-e 0+e],c3);plot([0 1 1 0 0],[0 0 1 1 0]);disp('weights');
  "IW{2,1}(299,:)'" : Constant  Value=[0.7575431891216286572898752638138830661773681640625;1.229213305581662307730539396288804709911346435546875;1.810083283739304160775418495177291333675384521484375;-0.1572310105014219361319049994563101790845394134521484375;-0.89747854557077177961588176913210190832614898681640625;-1.1192368173888407323346427801880054175853729248046875;0.7573089087472901770325961479102261364459991455078125;-1.79694214217461034621692306245677173137664794921875]
      mask Display: e = 0.06;c1 = [120 150 230]/255;c2 = ([120 150 230]+0)/383;c3 = ([120 150 230]+128)/383;patch([0 1 1 0],[0 0 1 1],c1);patch([0 1 1 1-e 1-e 0+e],[0 0 1 1-e 0+e 0+e],c2);patch([0 0 1 1-e 0+e 0+e],[0 1 1 1-e 1-e 0+e],c3);plot([0 1 1 0 0],[0 0 1 1 0]);disp('weights');
  "IW{2,1}(3,:)'" : Constant  Value=[-0.83690372965789172621242641980643384158611297607421875;-1.154914680191724496438610003679059445858001708984375;1.13904575215728431913930762675590813159942626953125;0.95361878259994081741268701080116443336009979248046875;1.0615310460876534737195697744027711451053619384765625;0.286424987747621262457187185646034777164459228515625;-1.672805025225078789929966660565696656703948974609375;1.6609915496172871218760747069609351456165313720703125]
      mask Display: e = 0.06;c1 = [120 150 230]/255;c2 = ([120 150 230]+0)/383;c3 = ([120 150 230]+128)/383;patch([0 1 1 0],[0 0 1 1],c1);patch([0 1 1 1-e 1-e 0+e],[0 0 1 1-e 0+e 0+e],c2);patch([0 0 1 1-e 0+e 0+e],[0 1 1 1-e 1-e 0+e],c3);plot([0 1 1 0 0],[0 0 1 1 0]);disp('weights');
  "IW{2,1}(30,:)'" : Constant  Value=[-0.8706022673904982855930256846477277576923370361328125;-0.0879880741568741242542017744199256412684917449951171875;-0.323123551430262445638419421811704523861408233642578125;2.02198320106408768737082937150262296199798583984375;-0.86868500420774619197317178986850194633007049560546875;1.5624300902894974196755129014491103589534759521484375;1.6535207444727422210206668751197867095470428466796875;0.363206518091484298338400549255311489105224609375]
      mask Display: e = 0.06;c1 = [120 150 230]/255;c2 = ([120 150 230]+0)/383;c3 = ([120 150 230]+128)/383;patch([0 1 1 0],[0 0 1 1],c1);patch([0 1 1 1-e 1-e 0+e],[0 0 1 1-e 0+e 0+e],c2);patch([0 0 1 1-e 0+e 0+e],[0 1 1 1-e 1-e 0+e],c3);plot([0 1 1 0 0],[0 0 1 1 0]);disp('weights');
  "IW{2,1}(300,:)'" : Constant  Value=[-0.4695024464110899575786106652230955660343170166015625;-1.203705732039551445922143102507106959819793701171875;1.5130380234864684307893867298844270408153533935546875;1.3198736861827431443572322677937336266040802001953125;0.94438292148976887840916560890036635100841522216796875;-1.257930292994181353805061007733456790447235107421875;0.6973943764304555426036813514656387269496917724609375;1.5243184165398451224149312110967002809047698974609375]
      mask Display: e = 0.06;c1 = [120 150 230]/255;c2 = ([120 150 230]+0)/383;c3 = ([120 150 230]+128)/383;patch([0 1 1 0],[0 0 1 1],c1);patch([0 1 1 1-e 1-e 0+e],[0 0 1 1-e 0+e 0+e],c2);patch([0 0 1 1-e 0+e 0+e],[0 1 1 1-e 1-e 0+e],c3);plot([0 1 1 0 0],[0 0 1 1 0]);disp('weights');
  "IW{2,1}(301,:)'" : Constant  Value=[1.4992730582447182374750127564766444265842437744140625;-1.171026328408421246507487012422643601894378662109375;-0.5802693343082570009983101044781506061553955078125;-0.265006801952717252479629905792535282671451568603515625;0.8986575966217895672372151238960213959217071533203125;-1.120628035919562393019077717326581478118896484375;0.0262365055607453843966592188508002436719834804534912109375;-2.2217585154337573527527638361789286136627197265625]
      mask Display: e = 0.06;c1 = [120 150 230]/255;c2 = ([120 150 230]+0)/383;c3 = ([120 150 230]+128)/383;patch([0 1 1 0],[0 0 1 1],c1);patch([0 1 1 1-e 1-e 0+e],[0 0 1 1-e 0+e 0+e],c2);patch([0 0 1 1-e 0+e 0+e],[0 1 1 1-e 1-e 0+e],c3);plot([0 1 1 0 0],[0 0 1 1 0]);disp('weights');
  "IW{2,1}(302,:)'" : Constant  Value=[0.21645160550166575585961936667445115745067596435546875;1.7280621165898637503488544098217971622943878173828125;-1.115894301542621036560376523993909358978271484375;-0.99211020457547594020297765382565557956695556640625;-0.460189482165866914353813399429782293736934661865234375;1.2553463408558072078591294484795071184635162353515625;0.97984291896522612841380350801046006381511688232421875;-1.7219603540277537145897213122225366532802581787109375]
      mask Display: e = 0.06;c1 = [120 150 230]/255;c2 = ([120 150 230]+0)/383;c3 = ([120 150 230]+128)/383;patch([0 1 1 0],[0 0 1 1],c1);patch([0 1 1 1-e 1-e 0+e],[0 0 1 1-e 0+e 0+e],c2);patch([0 0 1 1-e 0+e 0+e],[0 1 1 1-e 1-e 0+e],c3);plot([0 1 1 0 0],[0 0 1 1 0]);disp('weights');
  "IW{2,1}(303,:)'" : Constant  Value=[-1.577092748516073061892939222161658108234405517578125;1.0490463847864577306978617343702353537082672119140625;0.2235141932496018946086024925534729845821857452392578125;-1.4370937545338706708974996217875741422176361083984375;-0.320615855533113391917510170969762839376926422119140625;-1.4147879504585691989859697059728205204010009765625;1.202651104290481054448491704533807933330535888671875;-1.3977749395487675254656778633943758904933929443359375]
      mask Display: e = 0.06;c1 = [120 150 230]/255;c2 = ([120 150 230]+0)/383;c3 = ([120 150 230]+128)/383;patch([0 1 1 0],[0 0 1 1],c1);patch([0 1 1 1-e 1-e 0+e],[0 0 1 1-e 0+e 0+e],c2);patch([0 0 1 1-e 0+e 0+e],[0 1 1 1-e 1-e 0+e],c3);plot([0 1 1 0 0],[0 0 1 1 0]);disp('weights');
  "IW{2,1}(304,:)'" : Constant  Value=[0.95787182259439707099346605900791473686695098876953125;1.2051911870966500739399407393648289144039154052734375;1.175954113818607371655389215447939932346343994140625;-0.80872558624624779621825609865481965243816375732421875;-1.9341362336565512958230783624458126723766326904296875;-0.7913495011414168889274378670961596071720123291015625;-0.58319732273415747503264583428972400724887847900390625;-1.405435564894582878281426019384525716304779052734375]
      mask Display: e = 0.06;c1 = [120 150 230]/255;c2 = ([120 150 230]+0)/383;c3 = ([120 150 230]+128)/383;patch([0 1 1 0],[0 0 1 1],c1);patch([0 1 1 1-e 1-e 0+e],[0 0 1 1-e 0+e 0+e],c2);patch([0 0 1 1-e 0+e 0+e],[0 1 1 1-e 1-e 0+e],c3);plot([0 1 1 0 0],[0 0 1 1 0]);disp('weights');
  "IW{2,1}(305,:)'" : Constant  Value=[0.0232546618312756796231877132186127710156142711639404296875;-1.6267041491998106561567283279146067798137664794921875;-0.68505978158889624385352590252296067774295806884765625;0.600360426501180821645675678155384957790374755859375;-1.644927790605635209431056864559650421142578125;0.29752486775745634606238354535889811813831329345703125;2.061487220312472334882158975233323872089385986328125;-0.74776707636719985661244436414563097059726715087890625]
      mask Display: e = 0.06;c1 = [120 150 230]/255;c2 = ([120 150 230]+0)/383;c3 = ([120 150 230]+128)/383;patch([0 1 1 0],[0 0 1 1],c1);patch([0 1 1 1-e 1-e 0+e],[0 0 1 1-e 0+e 0+e],c2);patch([0 0 1 1-e 0+e 0+e],[0 1 1 1-e 1-e 0+e],c3);plot([0 1 1 0 0],[0 0 1 1 0]);disp('weights');
  "IW{2,1}(306,:)'" : Constant  Value=[0.307643507114700398563655880934675224125385284423828125;-1.7516940236946150211139183738850988447666168212890625;-1.339174217498975139051253790967166423797607421875;-0.50228666573348423884937119510141201317310333251953125;1.658098944714120559495995621546171605587005615234375;-0.954504314461473324371354465256445109844207763671875;1.3790483009797374069904662974295206367969512939453125;-0.5206775011140762909889190268586389720439910888671875]
      mask Display: e = 0.06;c1 = [120 150 230]/255;c2 = ([120 150 230]+0)/383;c3 = ([120 150 230]+128)/383;patch([0 1 1 0],[0 0 1 1],c1);patch([0 1 1 1-e 1-e 0+e],[0 0 1 1-e 0+e 0+e],c2);patch([0 0 1 1-e 0+e 0+e],[0 1 1 1-e 1-e 0+e],c3);plot([0 1 1 0 0],[0 0 1 1 0]);disp('weights');
  "IW{2,1}(307,:)'" : Constant  Value=[-2.036521733314567317307819394045509397983551025390625;-1.0843540474509556492677120331791229546070098876953125;-0.978043574355647482576614493154920637607574462890625;1.20291024816412317477443139068782329559326171875;0.07484893373486158074658902705778018571436405181884765625;-0.9633395431981062184689790228730998933315277099609375;1.218326453460640390602520710672251880168914794921875;-0.9428558183991169183713054735562764108180999755859375]
      mask Display: e = 0.06;c1 = [120 150 230]/255;c2 = ([120 150 230]+0)/383;c3 = ([120 150 230]+128)/383;patch([0 1 1 0],[0 0 1 1],c1);patch([0 1 1 1-e 1-e 0+e],[0 0 1 1-e 0+e 0+e],c2);patch([0 0 1 1-e 0+e 0+e],[0 1 1 1-e 1-e 0+e],c3);plot([0 1 1 0 0],[0 0 1 1 0]);disp('weights');
  "IW{2,1}(308,:)'" : Constant  Value=[-0.343697267399743100479980739692109636962413787841796875;-2.357305464479904077990113364649005234241485595703125;0.82850372760230717172902359379804693162441253662109375;-0.6411439272598438154915356790297664701938629150390625;0.08881403549962600674216872675970080308616161346435546875;-0.5011156454033380835966227095923386514186859130859375;1.820618658772904741027787167695350944995880126953125;-0.67047534773334305224778972842614166438579559326171875]
      mask Display: e = 0.06;c1 = [120 150 230]/255;c2 = ([120 150 230]+0)/383;c3 = ([120 150 230]+128)/383;patch([0 1 1 0],[0 0 1 1],c1);patch([0 1 1 1-e 1-e 0+e],[0 0 1 1-e 0+e 0+e],c2);patch([0 0 1 1-e 0+e 0+e],[0 1 1 1-e 1-e 0+e],c3);plot([0 1 1 0 0],[0 0 1 1 0]);disp('weights');
  "IW{2,1}(309,:)'" : Constant  Value=[-1.818679086724649618389548777486197650432586669921875;-0.0225100328944918652573914386039177770726382732391357421875;-1.2850894056110899743572417719406075775623321533203125;0.58506139016945468700470200928975827991962432861328125;0.49690343152257998582399523002095520496368408203125;-2.300348438279462559563626200542785227298736572265625;0.274003116541775504355626935648615472018718719482421875;-0.282474236572137382683678197281551547348499298095703125]
      mask Display: e = 0.06;c1 = [120 150 230]/255;c2 = ([120 150 230]+0)/383;c3 = ([120 150 230]+128)/383;patch([0 1 1 0],[0 0 1 1],c1);patch([0 1 1 1-e 1-e 0+e],[0 0 1 1-e 0+e 0+e],c2);patch([0 0 1 1-e 0+e 0+e],[0 1 1 1-e 1-e 0+e],c3);plot([0 1 1 0 0],[0 0 1 1 0]);disp('weights');
  "IW{2,1}(31,:)'" : Constant  Value=[-0.6778220352334505260927244307822547852993011474609375;-1.002948065510846920034282447886653244495391845703125;0.01407924362783327144887923765281811938621103763580322265625;-1.65265069497485228566802106797695159912109375;-1.8678963103245307397770602619857527315616607666015625;1.6781190401603034434430128385429270565509796142578125;0.4976509515009865936008282005786895751953125;0.052912337285146604504149081549257971346378326416015625]
      mask Display: e = 0.06;c1 = [120 150 230]/255;c2 = ([120 150 230]+0)/383;c3 = ([120 150 230]+128)/383;patch([0 1 1 0],[0 0 1 1],c1);patch([0 1 1 1-e 1-e 0+e],[0 0 1 1-e 0+e 0+e],c2);patch([0 0 1 1-e 0+e 0+e],[0 1 1 1-e 1-e 0+e],c3);plot([0 1 1 0 0],[0 0 1 1 0]);disp('weights');
  "IW{2,1}(310,:)'" : Constant  Value=[-0.9850737716051496395408548778505064547061920166015625;1.0636727649987989252622355706989765167236328125;-1.282862670891714795828875139704905450344085693359375;1.4226035718425353859828419444966129958629608154296875;1.3300607573897007540608683484606444835662841796875;-0.312953405537495898958155748914577998220920562744140625;-1.392344087340662728280449300655163824558258056640625;-1.0806948454210629773086793647962622344493865966796875]
      mask Display: e = 0.06;c1 = [120 150 230]/255;c2 = ([120 150 230]+0)/383;c3 = ([120 150 230]+128)/383;patch([0 1 1 0],[0 0 1 1],c1);patch([0 1 1 1-e 1-e 0+e],[0 0 1 1-e 0+e 0+e],c2);patch([0 0 1 1-e 0+e 0+e],[0 1 1 1-e 1-e 0+e],c3);plot([0 1 1 0 0],[0 0 1 1 0]);disp('weights');
  "IW{2,1}(311,:)'" : Constant  Value=[-0.49294553067137314439349893291364423930644989013671875;-1.9141901169723762876628825324587523937225341796875;-0.778270681123441221416214830242097377777099609375;-0.509205764484566003602594719268381595611572265625;-1.5227342365238640820024329514126293361186981201171875;1.628009143875833064640801239875145256519317626953125;1.15603318056876336328286924981512129306793212890625;0.031259373196099560221483670829911716282367706298828125]
      mask Display: e = 0.06;c1 = [120 150 230]/255;c2 = ([120 150 230]+0)/383;c3 = ([120 150 230]+128)/383;patch([0 1 1 0],[0 0 1 1],c1);patch([0 1 1 1-e 1-e 0+e],[0 0 1 1-e 0+e 0+e],c2);patch([0 0 1 1-e 0+e 0+e],[0 1 1 1-e 1-e 0+e],c3);plot([0 1 1 0 0],[0 0 1 1 0]);disp('weights');
  "IW{2,1}(312,:)'" : Constant  Value=[-0.92467661683877022671396161968004889786243438720703125;-0.10371882087682215978219346652622334659099578857421875;0.2472184768976093127701432194953667931258678436279296875;-1.636317894696662111897467184462584555149078369140625;1.3811472962270487929714590791263617575168609619140625;-0.33054749103647285135565425662207417190074920654296875;2.0426896508592786716462796903215348720550537109375;-1.2247719007705752947146038422943092882633209228515625]
      mask Display: e = 0.06;c1 = [120 150 230]/255;c2 = ([120 150 230]+0)/383;c3 = ([120 150 230]+128)/383;patch([0 1 1 0],[0 0 1 1],c1);patch([0 1 1 1-e 1-e 0+e],[0 0 1 1-e 0+e 0+e],c2);patch([0 0 1 1-e 0+e 0+e],[0 1 1 1-e 1-e 0+e],c3);plot([0 1 1 0 0],[0 0 1 1 0]);disp('weights');
  "IW{2,1}(313,:)'" : Constant  Value=[-1.6957828522094453571611438746913336217403411865234375;-0.8732839118050577109642063078354112803936004638671875;-0.677899071672815267675105133093893527984619140625;0.04858513887136466091742903472550096921622753143310546875;1.6130422595957825127044316104729659855365753173828125;1.062862964497595985591260614455677568912506103515625;-1.743369601694128245839010560302995145320892333984375;0.048899058400884438946309984430627082474529743194580078125]
      mask Display: e = 0.06;c1 = [120 150 230]/255;c2 = ([120 150 230]+0)/383;c3 = ([120 150 230]+128)/383;patch([0 1 1 0],[0 0 1 1],c1);patch([0 1 1 1-e 1-e 0+e],[0 0 1 1-e 0+e 0+e],c2);patch([0 0 1 1-e 0+e 0+e],[0 1 1 1-e 1-e 0+e],c3);plot([0 1 1 0 0],[0 0 1 1 0]);disp('weights');
  "IW{2,1}(314,:)'" : Constant  Value=[0.43872567744963408831182505309698171913623809814453125;0.99901835769378000140505946546909399330615997314453125;-1.553135455583668278478626234573312103748321533203125;-1.042050071829793811417630422511138021945953369140625;1.3456214852699586170814427532604895532131195068359375;1.496940581078169518747245092527009546756744384765625;-1.507263024349582369865174769074656069278717041015625;0.449444590311120772962993896726402454078197479248046875]
      mask Display: e = 0.06;c1 = [120 150 230]/255;c2 = ([120 150 230]+0)/383;c3 = ([120 150 230]+128)/383;patch([0 1 1 0],[0 0 1 1],c1);patch([0 1 1 1-e 1-e 0+e],[0 0 1 1-e 0+e 0+e],c2);patch([0 0 1 1-e 0+e 0+e],[0 1 1 1-e 1-e 0+e],c3);plot([0 1 1 0 0],[0 0 1 1 0]);disp('weights');
  "IW{2,1}(315,:)'" : Constant  Value=[1.0115042201612054473258694997639395296573638916015625;1.5366306570953611743135525102843530476093292236328125;-1.16260833460016232976386163500137627124786376953125;-0.9904503698687914248210972800734452903270721435546875;-0.73803809418303245593051542527973651885986328125;1.320787028949091723717401691828854382038116455078125;-0.97499989679716858592684047835064120590686798095703125;1.3644731164354368946334261636366136372089385986328125]
      mask Display: e = 0.06;c1 = [120 150 230]/255;c2 = ([120 150 230]+0)/383;c3 = ([120 150 230]+128)/383;patch([0 1 1 0],[0 0 1 1],c1);patch([0 1 1 1-e 1-e 0+e],[0 0 1 1-e 0+e 0+e],c2);patch([0 0 1 1-e 0+e 0+e],[0 1 1 1-e 1-e 0+e],c3);plot([0 1 1 0 0],[0 0 1 1 0]);disp('weights');
  "IW{2,1}(316,:)'" : Constant  Value=[-1.252813584453977835408977625775150954723358154296875;-0.5090112203525956058314250185503624379634857177734375;0.69399755402318152874840961885638535022735595703125;1.1407973848801227223503929053549654781818389892578125;1.87625240746523136436962886364199221134185791015625;0.76920158540545024994372624860261566936969757080078125;-0.1083699466948503109531287691424950025975704193115234375;-1.8186513669145492055889690163894556462764739990234375]
      mask Display: e = 0.06;c1 = [120 150 230]/255;c2 = ([120 150 230]+0)/383;c3 = ([120 150 230]+128)/383;patch([0 1 1 0],[0 0 1 1],c1);patch([0 1 1 1-e 1-e 0+e],[0 0 1 1-e 0+e 0+e],c2);patch([0 0 1 1-e 0+e 0+e],[0 1 1 1-e 1-e 0+e],c3);plot([0 1 1 0 0],[0 0 1 1 0]);disp('weights');
  "IW{2,1}(317,:)'" : Constant  Value=[1.099678212972654112178361174301244318485260009765625;-0.461170185635641993737721122670336626470088958740234375;1.750978350657032667214707544189877808094024658203125;-0.38955130020600459150870165103697218000888824462890625;-0.72022344640292790263202959977206774055957794189453125;1.636951316892007124437213860801421105861663818359375;-1.751085399497080086206324267550371587276458740234375;-0.53483708110640904020982588917831890285015106201171875]
      mask Display: e = 0.06;c1 = [120 150 230]/255;c2 = ([120 150 230]+0)/383;c3 = ([120 150 230]+128)/383;patch([0 1 1 0],[0 0 1 1],c1);patch([0 1 1 1-e 1-e 0+e],[0 0 1 1-e 0+e 0+e],c2);patch([0 0 1 1-e 0+e 0+e],[0 1 1 1-e 1-e 0+e],c3);plot([0 1 1 0 0],[0 0 1 1 0]);disp('weights');
  "IW{2,1}(318,:)'" : Constant  Value=[1.5417523631426341967909365848754532635211944580078125;-2.024876949691419181220908285467885434627532958984375;1.41026304797850787764446067740209400653839111328125;0.863613107959514625378005803213454782962799072265625;0.5790235228435047787343137315474450588226318359375;1.1363168558833718346789964925847016274929046630859375;-0.006183418124956588900198450886591672315262258052825927734375;0.49097130361616103666477783917798660695552825927734375]
      mask Display: e = 0.06;c1 = [120 150 230]/255;c2 = ([120 150 230]+0)/383;c3 = ([120 150 230]+128)/383;patch([0 1 1 0],[0 0 1 1],c1);patch([0 1 1 1-e 1-e 0+e],[0 0 1 1-e 0+e 0+e],c2);patch([0 0 1 1-e 0+e 0+e],[0 1 1 1-e 1-e 0+e],c3);plot([0 1 1 0 0],[0 0 1 1 0]);disp('weights');
  "IW{2,1}(319,:)'" : Constant  Value=[-1.8123440819783045441226931870914995670318603515625;-1.78110636927784593552814840222708880901336669921875;-0.296802646773347722497504719285643659532070159912109375;0.49775180415931974398091597322490997612476348876953125;-0.066135425957409010866427934161038137972354888916015625;1.4527647001454744302151311785564757883548736572265625;0.0210122335016035798049838234646813361905515193939208984375;1.5195235339768384807968004679423756897449493408203125]
      mask Display: e = 0.06;c1 = [120 150 230]/255;c2 = ([120 150 230]+0)/383;c3 = ([120 150 230]+128)/383;patch([0 1 1 0],[0 0 1 1],c1);patch([0 1 1 1-e 1-e 0+e],[0 0 1 1-e 0+e 0+e],c2);patch([0 0 1 1-e 0+e 0+e],[0 1 1 1-e 1-e 0+e],c3);plot([0 1 1 0 0],[0 0 1 1 0]);disp('weights');
  "IW{2,1}(32,:)'" : Constant  Value=[0.177210476594283294904386139023699797689914703369140625;1.0500285814146632645815770956687629222869873046875;-1.3050924530824890013036565505899488925933837890625;1.55692392218179787022336313384585082530975341796875;1.9328061547376675921583455419749952852725982666015625;-1.0011300751400040720540118854842148721218109130859375;1.063662721562024682242508788476698100566864013671875;-0.1671090707737801495103013849075068719685077667236328125]
      mask Display: e = 0.06;c1 = [120 150 230]/255;c2 = ([120 150 230]+0)/383;c3 = ([120 150 230]+128)/383;patch([0 1 1 0],[0 0 1 1],c1);patch([0 1 1 1-e 1-e 0+e],[0 0 1 1-e 0+e 0+e],c2);patch([0 0 1 1-e 0+e 0+e],[0 1 1 1-e 1-e 0+e],c3);plot([0 1 1 0 0],[0 0 1 1 0]);disp('weights');
  "IW{2,1}(320,:)'" : Constant  Value=[-0.844191671750298855414484933135099709033966064453125;-0.98194553653667970838370138153550215065479278564453125;1.4780105940430221522774445475079119205474853515625;-0.960600126189331771087154265842400491237640380859375;0.60400332325700067936935511170304380357265472412109375;-1.7417275014529158827514265794889070093631744384765625;1.4130636677642944842858696574694477021694183349609375;1.06547921441438386835898199933581054210662841796875]
      mask Display: e = 0.06;c1 = [120 150 230]/255;c2 = ([120 150 230]+0)/383;c3 = ([120 150 230]+128)/383;patch([0 1 1 0],[0 0 1 1],c1);patch([0 1 1 1-e 1-e 0+e],[0 0 1 1-e 0+e 0+e],c2);patch([0 0 1 1-e 0+e 0+e],[0 1 1 1-e 1-e 0+e],c3);plot([0 1 1 0 0],[0 0 1 1 0]);disp('weights');
  "IW{2,1}(321,:)'" : Constant  Value=[-1.64625721295164506585706476471386849880218505859375;-1.495058170556912813253802596591413021087646484375;-0.643205466600353492623298734542913734912872314453125;-0.53701532456692102623918572135153226554393768310546875;1.4916601893069680873082916150451637804508209228515625;-0.61602277182288045498381734432769007980823516845703125;-1.5856616773009084564449722165591083467006683349609375;0.60934455628117467629323300570831634104251861572265625]
      mask Display: e = 0.06;c1 = [120 150 230]/255;c2 = ([120 150 230]+0)/383;c3 = ([120 150 230]+128)/383;patch([0 1 1 0],[0 0 1 1],c1);patch([0 1 1 1-e 1-e 0+e],[0 0 1 1-e 0+e 0+e],c2);patch([0 0 1 1-e 0+e 0+e],[0 1 1 1-e 1-e 0+e],c3);plot([0 1 1 0 0],[0 0 1 1 0]);disp('weights');
  "IW{2,1}(322,:)'" : Constant  Value=[0.8984843155652983970327341012307442724704742431640625;-0.74012032252163428847069326366181485354900360107421875;0.245627681424364363582668602248304523527622222900390625;1.853171188690172499491382041014730930328369140625;1.4968259686539131525506718389806337654590606689453125;1.125733028011529857081995942280627787113189697265625;-1.251881118996162722822873547556810081005096435546875;-0.97813033057623766097776751848869025707244873046875]
      mask Display: e = 0.06;c1 = [120 150 230]/255;c2 = ([120 150 230]+0)/383;c3 = ([120 150 230]+128)/383;patch([0 1 1 0],[0 0 1 1],c1);patch([0 1 1 1-e 1-e 0+e],[0 0 1 1-e 0+e 0+e],c2);patch([0 0 1 1-e 0+e 0+e],[0 1 1 1-e 1-e 0+e],c3);plot([0 1 1 0 0],[0 0 1 1 0]);disp('weights');
  "IW{2,1}(323,:)'" : Constant  Value=[-0.167570785224088802944919507353915832936763763427734375;-1.3985166343418440337842412191093899309635162353515625;-0.60738873407524407443958125440985895693302154541015625;-0.14361192473872474995033599043381400406360626220703125;-0.99194312094749348407418665374279953539371490478515625;-1.751398493027971792201924472465179860591888427734375;1.2524876754701843584172138434951193630695343017578125;1.6926545467356988172724641117383725941181182861328125]
      mask Display: e = 0.06;c1 = [120 150 230]/255;c2 = ([120 150 230]+0)/383;c3 = ([120 150 230]+128)/383;patch([0 1 1 0],[0 0 1 1],c1);patch([0 1 1 1-e 1-e 0+e],[0 0 1 1-e 0+e 0+e],c2);patch([0 0 1 1-e 0+e 0+e],[0 1 1 1-e 1-e 0+e],c3);plot([0 1 1 0 0],[0 0 1 1 0]);disp('weights');
  "IW{2,1}(324,:)'" : Constant  Value=[1.3735780780273676437985841403133235871791839599609375;0.6611783672958992941204314774950034916400909423828125;-1.522300296614170544984290245338343083858489990234375;1.2218856458518743135499562413315288722515106201171875;-0.537835288144763001838555283029563724994659423828125;-0.419592181741024028429620784663711674511432647705078125;-1.788727238440078526338083975133486092090606689453125;1.2404240424056443004019456566311419010162353515625]
      mask Display: e = 0.06;c1 = [120 150 230]/255;c2 = ([120 150 230]+0)/383;c3 = ([120 150 230]+128)/383;patch([0 1 1 0],[0 0 1 1],c1);patch([0 1 1 1-e 1-e 0+e],[0 0 1 1-e 0+e 0+e],c2);patch([0 0 1 1-e 0+e 0+e],[0 1 1 1-e 1-e 0+e],c3);plot([0 1 1 0 0],[0 0 1 1 0]);disp('weights');
  "IW{2,1}(325,:)'" : Constant  Value=[0.9904275298239475500139405994559638202190399169921875;1.562865104975433183653876767493784427642822265625;-1.0836385414812974570253345518722198903560638427734375;1.5083182315329037859186200876138173043727874755859375;0.2167450835400050179746500589317292906343936920166015625;-0.4977926766720524032194816754781641066074371337890625;-1.156264904238256452373434512992389500141143798828125;1.55923675124961480520369150326587259769439697265625]
      mask Display: e = 0.06;c1 = [120 150 230]/255;c2 = ([120 150 230]+0)/383;c3 = ([120 150 230]+128)/383;patch([0 1 1 0],[0 0 1 1],c1);patch([0 1 1 1-e 1-e 0+e],[0 0 1 1-e 0+e 0+e],c2);patch([0 0 1 1-e 0+e 0+e],[0 1 1 1-e 1-e 0+e],c3);plot([0 1 1 0 0],[0 0 1 1 0]);disp('weights');
  "IW{2,1}(326,:)'" : Constant  Value=[-0.3394698356902818847657954393071122467517852783203125;1.254735850017049347826514349435456097126007080078125;-0.2465374496213206534367401445706491358578205108642578125;-0.8740890755012096224874085237388499081134796142578125;0.485580537707730186536281280496041290462017059326171875;1.9169916556036536992024821302038617432117462158203125;-2.131079188199580531914989478536881506443023681640625;-0.466929236576190176410960930297733284533023834228515625]
      mask Display: e = 0.06;c1 = [120 150 230]/255;c2 = ([120 150 230]+0)/383;c3 = ([120 150 230]+128)/383;patch([0 1 1 0],[0 0 1 1],c1);patch([0 1 1 1-e 1-e 0+e],[0 0 1 1-e 0+e 0+e],c2);patch([0 0 1 1-e 0+e 0+e],[0 1 1 1-e 1-e 0+e],c3);plot([0 1 1 0 0],[0 0 1 1 0]);disp('weights');
  "IW{2,1}(327,:)'" : Constant  Value=[-0.27202773816425074304703457528376020491123199462890625;1.5046072601150093372979199557448737323284149169921875;1.4218117962618761485060758786858059465885162353515625;0.478585925259448818902541233910596929490566253662109375;0.0025322775019821423640731250515045758220367133617401123046875;0.61421035017912528619632439585984684526920318603515625;1.6447229054945438075918673348496668040752410888671875;1.8277378348829158571930975085706450045108795166015625]
      mask Display: e = 0.06;c1 = [120 150 230]/255;c2 = ([120 150 230]+0)/383;c3 = ([120 150 230]+128)/383;patch([0 1 1 0],[0 0 1 1],c1);patch([0 1 1 1-e 1-e 0+e],[0 0 1 1-e 0+e 0+e],c2);patch([0 0 1 1-e 0+e 0+e],[0 1 1 1-e 1-e 0+e],c3);plot([0 1 1 0 0],[0 0 1 1 0]);disp('weights');
  "IW{2,1}(328,:)'" : Constant  Value=[-1.999923474432578895942924646078608930110931396484375;1.1960060721962284535635490101412869989871978759765625;-0.451012543585936287460214089151122607290744781494140625;-1.6319193363516248940214836693485267460346221923828125;1.59291702470226947951914553414098918437957763671875;0.37426920215524750457092295619077049195766448974609375;0.302030853333788484871291757372091524302959442138671875;0.10971960402364666631314094047411344945430755615234375]
      mask Display: e = 0.06;c1 = [120 150 230]/255;c2 = ([120 150 230]+0)/383;c3 = ([120 150 230]+128)/383;patch([0 1 1 0],[0 0 1 1],c1);patch([0 1 1 1-e 1-e 0+e],[0 0 1 1-e 0+e 0+e],c2);patch([0 0 1 1-e 0+e 0+e],[0 1 1 1-e 1-e 0+e],c3);plot([0 1 1 0 0],[0 0 1 1 0]);disp('weights');
  "IW{2,1}(329,:)'" : Constant  Value=[-1.479702945174603545552827199571765959262847900390625;-0.6529372235373795962942722326260991394519805908203125;-0.85628932084014663939086631216923706233501434326171875;-1.1805605824152942684435174669488333165645599365234375;-1.19210241127462612809040365391410887241363525390625;1.3846333216222108664084089468815363943576812744140625;1.3773364506237542048694422192056663334369659423828125;1.120877854225029945922642582445405423641204833984375]
      mask Display: e = 0.06;c1 = [120 150 230]/255;c2 = ([120 150 230]+0)/383;c3 = ([120 150 230]+128)/383;patch([0 1 1 0],[0 0 1 1],c1);patch([0 1 1 1-e 1-e 0+e],[0 0 1 1-e 0+e 0+e],c2);patch([0 0 1 1-e 0+e 0+e],[0 1 1 1-e 1-e 0+e],c3);plot([0 1 1 0 0],[0 0 1 1 0]);disp('weights');
  "IW{2,1}(33,:)'" : Constant  Value=[1.2494120483460111614704146631993353366851806640625;0.287878839631612704064167473916313610970973968505859375;0.24359823614352593690313142360537312924861907958984375;1.6376719827248376049055877956561744213104248046875;-1.4219777775836615063553836080245673656463623046875;-1.353914885936317258341432534507475793361663818359375;-1.3913722165907049799216110841371119022369384765625;-0.91803628824360450355612783823744393885135650634765625]
      mask Display: e = 0.06;c1 = [120 150 230]/255;c2 = ([120 150 230]+0)/383;c3 = ([120 150 230]+128)/383;patch([0 1 1 0],[0 0 1 1],c1);patch([0 1 1 1-e 1-e 0+e],[0 0 1 1-e 0+e 0+e],c2);patch([0 0 1 1-e 0+e 0+e],[0 1 1 1-e 1-e 0+e],c3);plot([0 1 1 0 0],[0 0 1 1 0]);disp('weights');
  "IW{2,1}(330,:)'" : Constant  Value=[1.0766797906041472021598792707663960754871368408203125;-1.7381666274310252351398276005056686699390411376953125;1.3175144936303564424662226883810944855213165283203125;-0.556617879327877318473838386125862598419189453125;-1.3710987329491928221614216454327106475830078125;0.295867087352674362765725391000160016119480133056640625;-0.55340509534196147267692822424578480422496795654296875;1.6067994388926407633988446832518093287944793701171875]
      mask Display: e = 0.06;c1 = [120 150 230]/255;c2 = ([120 150 230]+0)/383;c3 = ([120 150 230]+128)/383;patch([0 1 1 0],[0 0 1 1],c1);patch([0 1 1 1-e 1-e 0+e],[0 0 1 1-e 0+e 0+e],c2);patch([0 0 1 1-e 0+e 0+e],[0 1 1 1-e 1-e 0+e],c3);plot([0 1 1 0 0],[0 0 1 1 0]);disp('weights');
  "IW{2,1}(331,:)'" : Constant  Value=[1.5531494368444602738321691504097543656826019287109375;-0.52600393510336773683633282416849397122859954833984375;1.1315824695405958255634004672174341976642608642578125;-1.7522851156241958658910107260453514754772186279296875;0.513698793222964855686996088479645550251007080078125;-1.7901392409256271509576663447660394012928009033203125;-0.58220148229831913955223399170790798962116241455078125;0.29789888709788192588945321404025889933109283447265625]
      mask Display: e = 0.06;c1 = [120 150 230]/255;c2 = ([120 150 230]+0)/383;c3 = ([120 150 230]+128)/383;patch([0 1 1 0],[0 0 1 1],c1);patch([0 1 1 1-e 1-e 0+e],[0 0 1 1-e 0+e 0+e],c2);patch([0 0 1 1-e 0+e 0+e],[0 1 1 1-e 1-e 0+e],c3);plot([0 1 1 0 0],[0 0 1 1 0]);disp('weights');
  "IW{2,1}(332,:)'" : Constant  Value=[-1.0685557929594065029732519178651273250579833984375;1.475943755352597808183645611279644072055816650390625;-2.093641897866491685675782719044946134090423583984375;-0.303015148006441137340516434051096439361572265625;-1.6228549922897166357671494552050717175006866455078125;0.87317314872762963329222429820219986140727996826171875;-0.278875637707257151287620899893227033317089080810546875;0.2022082775511854502159536650651716627180576324462890625]
      mask Display: e = 0.06;c1 = [120 150 230]/255;c2 = ([120 150 230]+0)/383;c3 = ([120 150 230]+128)/383;patch([0 1 1 0],[0 0 1 1],c1);patch([0 1 1 1-e 1-e 0+e],[0 0 1 1-e 0+e 0+e],c2);patch([0 0 1 1-e 0+e 0+e],[0 1 1 1-e 1-e 0+e],c3);plot([0 1 1 0 0],[0 0 1 1 0]);disp('weights');
  "IW{2,1}(333,:)'" : Constant  Value=[1.579881782238048426592058604001067578792572021484375;2.0357366684869493411724761244840919971466064453125;-0.1261237810290510019672893804454361088573932647705078125;0.251518120290028457386455329469754360616207122802734375;1.7507872447040175867272182586020790040493011474609375;-0.1459670680179582513691372014363878406584262847900390625;1.056676422111010094084804222802631556987762451171875;0.60967567119986754153870833761175163090229034423828125]
      mask Display: e = 0.06;c1 = [120 150 230]/255;c2 = ([120 150 230]+0)/383;c3 = ([120 150 230]+128)/383;patch([0 1 1 0],[0 0 1 1],c1);patch([0 1 1 1-e 1-e 0+e],[0 0 1 1-e 0+e 0+e],c2);patch([0 0 1 1-e 0+e 0+e],[0 1 1 1-e 1-e 0+e],c3);plot([0 1 1 0 0],[0 0 1 1 0]);disp('weights');
  "IW{2,1}(334,:)'" : Constant  Value=[-0.398544097210651815377246975913294591009616851806640625;-0.357161321328545666720089002410531975328922271728515625;-1.5457317712648006580167248102952726185321807861328125;2.01889532100363755517946628970094025135040283203125;-1.3232353548925541719682996699702925980091094970703125;0.55625688761028058149094022155622951686382293701171875;0.80061774410786601396949890840915031731128692626953125;1.3822286057742936282721757379476912319660186767578125]
      mask Display: e = 0.06;c1 = [120 150 230]/255;c2 = ([120 150 230]+0)/383;c3 = ([120 150 230]+128)/383;patch([0 1 1 0],[0 0 1 1],c1);patch([0 1 1 1-e 1-e 0+e],[0 0 1 1-e 0+e 0+e],c2);patch([0 0 1 1-e 0+e 0+e],[0 1 1 1-e 1-e 0+e],c3);plot([0 1 1 0 0],[0 0 1 1 0]);disp('weights');
  "IW{2,1}(335,:)'" : Constant  Value=[1.3915244497898615616549022888648323714733123779296875;-0.65843048318107399996534923047875054180622100830078125;1.8899536565441066304771311479271389544010162353515625;-1.34721006825003097873150181840173900127410888671875;0.63905442969153425369910337394685484468936920166015625;1.162519409279834547987775295041501522064208984375;1.20876343462911250981051125563681125640869140625;-0.391415606203912636029684790628380142152309417724609375]
      mask Display: e = 0.06;c1 = [120 150 230]/255;c2 = ([120 150 230]+0)/383;c3 = ([120 150 230]+128)/383;patch([0 1 1 0],[0 0 1 1],c1);patch([0 1 1 1-e 1-e 0+e],[0 0 1 1-e 0+e 0+e],c2);patch([0 0 1 1-e 0+e 0+e],[0 1 1 1-e 1-e 0+e],c3);plot([0 1 1 0 0],[0 0 1 1 0]);disp('weights');
  "IW{2,1}(336,:)'" : Constant  Value=[-1.8166661313058403148801289717084728181362152099609375;0.08298824226823194039059927717971731908619403839111328125;-2.244496578460958513545620007789693772792816162109375;0.85444599734380755062801426902296952903270721435546875;-0.28776214096457508606619057900388725101947784423828125;-0.69621027307144423001972199926967732608318328857421875;-1.1238186527095239686246941346325911581516265869140625;0.2916882721366407249519170363782905042171478271484375]
      mask Display: e = 0.06;c1 = [120 150 230]/255;c2 = ([120 150 230]+0)/383;c3 = ([120 150 230]+128)/383;patch([0 1 1 0],[0 0 1 1],c1);patch([0 1 1 1-e 1-e 0+e],[0 0 1 1-e 0+e 0+e],c2);patch([0 0 1 1-e 0+e 0+e],[0 1 1 1-e 1-e 0+e],c3);plot([0 1 1 0 0],[0 0 1 1 0]);disp('weights');
  "IW{2,1}(337,:)'" : Constant  Value=[-1.4141053692286640330877389715169556438922882080078125;0.85210662819332971817942734560347162187099456787109375;1.61114488493269991664647022844292223453521728515625;-1.673795471202967899415625652181915938854217529296875;0.103128779979821116885574383559287525713443756103515625;1.213213129005425106043958294321782886981964111328125;-0.70526865711366137912108342788997106254100799560546875;-1.0948324739231483082591012134798802435398101806640625]
      mask Display: e = 0.06;c1 = [120 150 230]/255;c2 = ([120 150 230]+0)/383;c3 = ([120 150 230]+128)/383;patch([0 1 1 0],[0 0 1 1],c1);patch([0 1 1 1-e 1-e 0+e],[0 0 1 1-e 0+e 0+e],c2);patch([0 0 1 1-e 0+e 0+e],[0 1 1 1-e 1-e 0+e],c3);plot([0 1 1 0 0],[0 0 1 1 0]);disp('weights');
  "IW{2,1}(338,:)'" : Constant  Value=[0.85287987537984399910584443205152638256549835205078125;0.222141005420062709330153438713750801980495452880859375;-1.094118106837308257439644876285456120967864990234375;-1.396982719757624114009786353562958538532257080078125;-0.641183165889521067271061838255263864994049072265625;0.9861098405534118871429427599650807678699493408203125;0.71789827648489878963999899497139267623424530029296875;-2.3151699172427218087477740482427179813385009765625]
      mask Display: e = 0.06;c1 = [120 150 230]/255;c2 = ([120 150 230]+0)/383;c3 = ([120 150 230]+128)/383;patch([0 1 1 0],[0 0 1 1],c1);patch([0 1 1 1-e 1-e 0+e],[0 0 1 1-e 0+e 0+e],c2);patch([0 0 1 1-e 0+e 0+e],[0 1 1 1-e 1-e 0+e],c3);plot([0 1 1 0 0],[0 0 1 1 0]);disp('weights');
  "IW{2,1}(339,:)'" : Constant  Value=[0.0299258888866020568431114412533133872784674167633056640625;0.6288014167188240577388569363392889499664306640625;0.45943821790212047151413798928842879831790924072265625;1.70520342090470666818191602942533791065216064453125;1.25440801270502522157812563818879425525665283203125;-0.452026007497583426353315871892846189439296722412109375;1.50215511689706016085210649180226027965545654296875;1.8461981442814912046657127575599588453769683837890625]
      mask Display: e = 0.06;c1 = [120 150 230]/255;c2 = ([120 150 230]+0)/383;c3 = ([120 150 230]+128)/383;patch([0 1 1 0],[0 0 1 1],c1);patch([0 1 1 1-e 1-e 0+e],[0 0 1 1-e 0+e 0+e],c2);patch([0 0 1 1-e 0+e 0+e],[0 1 1 1-e 1-e 0+e],c3);plot([0 1 1 0 0],[0 0 1 1 0]);disp('weights');
  "IW{2,1}(34,:)'" : Constant  Value=[1.213900126441318061409901929437182843685150146484375;1.7238542101994112076823739698738791048526763916015625;-0.1746306976326444659886050203567720018327236175537109375;-1.88977765985373924451096172560937702655792236328125;-0.76282624358894890459481530342600308358669281005859375;-1.205401844755503049100298085249960422515869140625;0.92038218572006569306864776081056334078311920166015625;0.449794483927468180528563834741362370550632476806640625]
      mask Display: e = 0.06;c1 = [120 150 230]/255;c2 = ([120 150 230]+0)/383;c3 = ([120 150 230]+128)/383;patch([0 1 1 0],[0 0 1 1],c1);patch([0 1 1 1-e 1-e 0+e],[0 0 1 1-e 0+e 0+e],c2);patch([0 0 1 1-e 0+e 0+e],[0 1 1 1-e 1-e 0+e],c3);plot([0 1 1 0 0],[0 0 1 1 0]);disp('weights');
  "IW{2,1}(340,:)'" : Constant  Value=[1.343793774226882842270924811600707471370697021484375;1.0243751831023983900337270824820734560489654541015625;-0.86204652563295269818155475149978883564472198486328125;1.373312952537015352305616033845581114292144775390625;-1.463855390721494842409811099059879779815673828125;-1.0856125688863522693594632073654793202877044677734375;-1.482024293011354298954529440379701554775238037109375;0.3351079713640741086777552482089959084987640380859375]
      mask Display: e = 0.06;c1 = [120 150 230]/255;c2 = ([120 150 230]+0)/383;c3 = ([120 150 230]+128)/383;patch([0 1 1 0],[0 0 1 1],c1);patch([0 1 1 1-e 1-e 0+e],[0 0 1 1-e 0+e 0+e],c2);patch([0 0 1 1-e 0+e 0+e],[0 1 1 1-e 1-e 0+e],c3);plot([0 1 1 0 0],[0 0 1 1 0]);disp('weights');
  "IW{2,1}(341,:)'" : Constant  Value=[-0.187709115424161632201816019005491398274898529052734375;0.65100924840334728482815762617974542081356048583984375;0.394479318765612541053400263990624807775020599365234375;-1.2595712306562865112624649555073119699954986572265625;1.684708111095214011498910622322000563144683837890625;-1.7258598148083741374847477345610968768596649169921875;-0.78368369488468692107829838278121314942836761474609375;1.542696178368702764061026755371131002902984619140625]
      mask Display: e = 0.06;c1 = [120 150 230]/255;c2 = ([120 150 230]+0)/383;c3 = ([120 150 230]+128)/383;patch([0 1 1 0],[0 0 1 1],c1);patch([0 1 1 1-e 1-e 0+e],[0 0 1 1-e 0+e 0+e],c2);patch([0 0 1 1-e 0+e 0+e],[0 1 1 1-e 1-e 0+e],c3);plot([0 1 1 0 0],[0 0 1 1 0]);disp('weights');
  "IW{2,1}(342,:)'" : Constant  Value=[0.05707043076651245605557249973571742884814739227294921875;1.5587860693942647838383663838612847030162811279296875;0.70455050763422855109041620380594395101070404052734375;-0.061032667590735799334478173250317922793328762054443359375;-1.845980234884216475421681025181896984577178955078125;1.4360139740494746174448437159298919141292572021484375;-0.1793906075291699375728882159819477237761020660400390625;1.5498685444472724004327801594627089798450469970703125]
      mask Display: e = 0.06;c1 = [120 150 230]/255;c2 = ([120 150 230]+0)/383;c3 = ([120 150 230]+128)/383;patch([0 1 1 0],[0 0 1 1],c1);patch([0 1 1 1-e 1-e 0+e],[0 0 1 1-e 0+e 0+e],c2);patch([0 0 1 1-e 0+e 0+e],[0 1 1 1-e 1-e 0+e],c3);plot([0 1 1 0 0],[0 0 1 1 0]);disp('weights');
  "IW{2,1}(343,:)'" : Constant  Value=[0.01299521487245316499203884319513235823251307010650634765625;0.69064447679400287061213248307467438280582427978515625;-0.62992828300395442564507675342611037194728851318359375;-0.01378992480848185986364029531614505685865879058837890625;-2.19202318727702749612262778100557625293731689453125;-1.8941321084006370600860691411071456968784332275390625;1.0727714923196141061367825386696495115756988525390625;-0.80202805255789877403316268100752495229244232177734375]
      mask Display: e = 0.06;c1 = [120 150 230]/255;c2 = ([120 150 230]+0)/383;c3 = ([120 150 230]+128)/383;patch([0 1 1 0],[0 0 1 1],c1);patch([0 1 1 1-e 1-e 0+e],[0 0 1 1-e 0+e 0+e],c2);patch([0 0 1 1-e 0+e 0+e],[0 1 1 1-e 1-e 0+e],c3);plot([0 1 1 0 0],[0 0 1 1 0]);disp('weights');
  "IW{2,1}(344,:)'" : Constant  Value=[-1.3789348916959649482549821186694316565990447998046875;0.367087657355373409018284291960299015045166015625;-0.74369337219250331028064238125807605683803558349609375;0.3491050793878542890524840913712978363037109375;1.2428649878521389471330849119112826883792877197265625;-0.3774256204809542936118305078707635402679443359375;-2.45015987121840783657944484730251133441925048828125;-0.7357793870233784172540936197037808597087860107421875]
      mask Display: e = 0.06;c1 = [120 150 230]/255;c2 = ([120 150 230]+0)/383;c3 = ([120 150 230]+128)/383;patch([0 1 1 0],[0 0 1 1],c1);patch([0 1 1 1-e 1-e 0+e],[0 0 1 1-e 0+e 0+e],c2);patch([0 0 1 1-e 0+e 0+e],[0 1 1 1-e 1-e 0+e],c3);plot([0 1 1 0 0],[0 0 1 1 0]);disp('weights');
  "IW{2,1}(345,:)'" : Constant  Value=[-0.76788470987143042645328705475549213588237762451171875;-0.778209568737224355317039226065389811992645263671875;-1.6111873877225131312940220595919527113437652587890625;-0.43768450535890346397849270942970179021358489990234375;1.9529040669453754386353239169693551957607269287109375;-0.438607135529375635751847539722803048789501190185546875;-1.4115727923338325933144687951426021754741668701171875;-1.051192119071858943613051451393403112888336181640625]
      mask Display: e = 0.06;c1 = [120 150 230]/255;c2 = ([120 150 230]+0)/383;c3 = ([120 150 230]+128)/383;patch([0 1 1 0],[0 0 1 1],c1);patch([0 1 1 1-e 1-e 0+e],[0 0 1 1-e 0+e 0+e],c2);patch([0 0 1 1-e 0+e 0+e],[0 1 1 1-e 1-e 0+e],c3);plot([0 1 1 0 0],[0 0 1 1 0]);disp('weights');
  "IW{2,1}(346,:)'" : Constant  Value=[1.0190115534627863791428126205573789775371551513671875;0.77702932715418848719224342858069576323032379150390625;-1.269447042200763764441262537729926407337188720703125;-1.53396547011438588725695808534510433673858642578125;-1.03391795301536948414877770119346678256988525390625;1.1232138095856025739038841493311338126659393310546875;0.79007677707643597653230926880496554076671600341796875;1.5195545004477895023597966428496874868869781494140625]
      mask Display: e = 0.06;c1 = [120 150 230]/255;c2 = ([120 150 230]+0)/383;c3 = ([120 150 230]+128)/383;patch([0 1 1 0],[0 0 1 1],c1);patch([0 1 1 1-e 1-e 0+e],[0 0 1 1-e 0+e 0+e],c2);patch([0 0 1 1-e 0+e 0+e],[0 1 1 1-e 1-e 0+e],c3);plot([0 1 1 0 0],[0 0 1 1 0]);disp('weights');
  "IW{2,1}(347,:)'" : Constant  Value=[-1.8035523244645459417512256550253368914127349853515625;-0.67300531404054309003726075388840399682521820068359375;0.509404826602606330965272718458436429500579833984375;0.023705682899657347373345572805192205123603343963623046875;1.3847741620540954254892085373285226523876190185546875;1.725509778022205065184380146092735230922698974609375;-0.67855458689826708695846946284291334450244903564453125;1.331839452410927382430827492498792707920074462890625]
      mask Display: e = 0.06;c1 = [120 150 230]/255;c2 = ([120 150 230]+0)/383;c3 = ([120 150 230]+128)/383;patch([0 1 1 0],[0 0 1 1],c1);patch([0 1 1 1-e 1-e 0+e],[0 0 1 1-e 0+e 0+e],c2);patch([0 0 1 1-e 0+e 0+e],[0 1 1 1-e 1-e 0+e],c3);plot([0 1 1 0 0],[0 0 1 1 0]);disp('weights');
  "IW{2,1}(348,:)'" : Constant  Value=[1.7018031849570023350537439910112880170345306396484375;1.710655419728059900563721384969539940357208251953125;-1.01060015145811465941960705094970762729644775390625;0.693583476488031980267123799421824514865875244140625;0.298171104644878337541769042218220420181751251220703125;1.78321994951979068133596229017712175846099853515625;-0.45025205185692251941276254001422785222530364990234375;-0.285276949762296505586078865235322155058383941650390625]
      mask Display: e = 0.06;c1 = [120 150 230]/255;c2 = ([120 150 230]+0)/383;c3 = ([120 150 230]+128)/383;patch([0 1 1 0],[0 0 1 1],c1);patch([0 1 1 1-e 1-e 0+e],[0 0 1 1-e 0+e 0+e],c2);patch([0 0 1 1-e 0+e 0+e],[0 1 1 1-e 1-e 0+e],c3);plot([0 1 1 0 0],[0 0 1 1 0]);disp('weights');
  "IW{2,1}(349,:)'" : Constant  Value=[0.4126768777415581457290727485087700188159942626953125;0.4246558500657655610410756708006374537944793701171875;-1.4873384012689305766485858839587308466434478759765625;1.4594915595233708405231709548388607800006866455078125;-0.03419641500078811346963192363546113483607769012451171875;-1.3099991530491272850866835142369382083415985107421875;-1.0283719201469818660399369036895222961902618408203125;-1.8892614723858851544235903929802589118480682373046875]
      mask Display: e = 0.06;c1 = [120 150 230]/255;c2 = ([120 150 230]+0)/383;c3 = ([120 150 230]+128)/383;patch([0 1 1 0],[0 0 1 1],c1);patch([0 1 1 1-e 1-e 0+e],[0 0 1 1-e 0+e 0+e],c2);patch([0 0 1 1-e 0+e 0+e],[0 1 1 1-e 1-e 0+e],c3);plot([0 1 1 0 0],[0 0 1 1 0]);disp('weights');
  "IW{2,1}(35,:)'" : Constant  Value=[0.421311053053571082926964663784019649028778076171875;-1.146135993313003087479273744975216686725616455078125;0.355451480360427340965401299399673007428646087646484375;-1.9731950793423804757509287810535170137882232666015625;-1.05439733869894691764557137503288686275482177734375;-1.9662161986900874577344211502349935472011566162109375;-0.73130361183941083869086696722661145031452178955078125;0.037217693981605688702263279310500365681946277618408203125]
      mask Display: e = 0.06;c1 = [120 150 230]/255;c2 = ([120 150 230]+0)/383;c3 = ([120 150 230]+128)/383;patch([0 1 1 0],[0 0 1 1],c1);patch([0 1 1 1-e 1-e 0+e],[0 0 1 1-e 0+e 0+e],c2);patch([0 0 1 1-e 0+e 0+e],[0 1 1 1-e 1-e 0+e],c3);plot([0 1 1 0 0],[0 0 1 1 0]);disp('weights');
  "IW{2,1}(350,:)'" : Constant  Value=[0.1585867768093802976370199075972777791321277618408203125;0.615701024201391167167685125605203211307525634765625;0.74866841188485222513548933420679531991481781005859375;-0.49537842307587987011885388710652478039264678955078125;-0.94143284430279361441051833025994710624217987060546875;-2.32824484848259150027161012985743582248687744140625;-1.865354136064464984912092404556460678577423095703125;0.10930195192903513490279010511585511267185211181640625]
      mask Display: e = 0.06;c1 = [120 150 230]/255;c2 = ([120 150 230]+0)/383;c3 = ([120 150 230]+128)/383;patch([0 1 1 0],[0 0 1 1],c1);patch([0 1 1 1-e 1-e 0+e],[0 0 1 1-e 0+e 0+e],c2);patch([0 0 1 1-e 0+e 0+e],[0 1 1 1-e 1-e 0+e],c3);plot([0 1 1 0 0],[0 0 1 1 0]);disp('weights');
  "IW{2,1}(351,:)'" : Constant  Value=[-1.242865874852193908139952327474020421504974365234375;-0.179851736345203516709290170183521695435047149658203125;-1.8747080505835416186499742252635769546031951904296875;0.85272596229702013470586052790167741477489471435546875;-0.5936433380912677915119957106071524322032928466796875;1.59415104941349294875863051856867969036102294921875;-0.25919553207987544585222394744050689041614532470703125;-1.5258015696692777130039075927925296127796173095703125]
      mask Display: e = 0.06;c1 = [120 150 230]/255;c2 = ([120 150 230]+0)/383;c3 = ([120 150 230]+128)/383;patch([0 1 1 0],[0 0 1 1],c1);patch([0 1 1 1-e 1-e 0+e],[0 0 1 1-e 0+e 0+e],c2);patch([0 0 1 1-e 0+e 0+e],[0 1 1 1-e 1-e 0+e],c3);plot([0 1 1 0 0],[0 0 1 1 0]);disp('weights');
  "IW{2,1}(352,:)'" : Constant  Value=[1.4948148900692610485663180952542461454868316650390625;-0.1482291862432829898654773614907753653824329376220703125;-0.89540931458373040907616768890875391662120819091796875;0.58085535563851464768703181107412092387676239013671875;-1.5706144603045195662360811184043996036052703857421875;-0.2369759154145947566139085438408073969185352325439453125;-0.2399287583522483335851660513071692548692226409912109375;2.268461431448778764519147443934343755245208740234375]
      mask Display: e = 0.06;c1 = [120 150 230]/255;c2 = ([120 150 230]+0)/383;c3 = ([120 150 230]+128)/383;patch([0 1 1 0],[0 0 1 1],c1);patch([0 1 1 1-e 1-e 0+e],[0 0 1 1-e 0+e 0+e],c2);patch([0 0 1 1-e 0+e 0+e],[0 1 1 1-e 1-e 0+e],c3);plot([0 1 1 0 0],[0 0 1 1 0]);disp('weights');
  "IW{2,1}(353,:)'" : Constant  Value=[1.4688012404645991448859376760083250701427459716796875;0.330693624535953134557786370351095683872699737548828125;0.92284151855501106442858372247428633272647857666015625;-0.443723850889678583797604005667380988597869873046875;1.71356791934530772181233260198496282100677490234375;-1.0283888840924435559287530850269831717014312744140625;-1.5281726580370802448527456363081000745296478271484375;-1.3644647988168878693926444611861370503902435302734375]
      mask Display: e = 0.06;c1 = [120 150 230]/255;c2 = ([120 150 230]+0)/383;c3 = ([120 150 230]+128)/383;patch([0 1 1 0],[0 0 1 1],c1);patch([0 1 1 1-e 1-e 0+e],[0 0 1 1-e 0+e 0+e],c2);patch([0 0 1 1-e 0+e 0+e],[0 1 1 1-e 1-e 0+e],c3);plot([0 1 1 0 0],[0 0 1 1 0]);disp('weights');
  "IW{2,1}(354,:)'" : Constant  Value=[0.86861990587902493388128277729265391826629638671875;0.321306095250735668233943442828604020178318023681640625;0.08106029031569016163327745516653521917760372161865234375;1.8601477073267338457895903047756291925907135009765625;1.8180876481239300890280219391570426523685455322265625;1.27802338945291893423927831463515758514404296875;-1.2923676080343156069574206412653438746929168701171875;-0.01096967278180301270940066871162343886680901050567626953125]
      mask Display: e = 0.06;c1 = [120 150 230]/255;c2 = ([120 150 230]+0)/383;c3 = ([120 150 230]+128)/383;patch([0 1 1 0],[0 0 1 1],c1);patch([0 1 1 1-e 1-e 0+e],[0 0 1 1-e 0+e 0+e],c2);patch([0 0 1 1-e 0+e 0+e],[0 1 1 1-e 1-e 0+e],c3);plot([0 1 1 0 0],[0 0 1 1 0]);disp('weights');
  "IW{2,1}(355,:)'" : Constant  Value=[-0.4269902444553912435054598972783423960208892822265625;-1.1283321328502549096839402409386821091175079345703125;1.4668785624222644425884709562524221837520599365234375;-0.6470754976427490756663019055849872529506683349609375;-0.79438639400969901505078496484202332794666290283203125;2.1334673700290256448397485655732452869415283203125;0.55664317441234534289407065443811006844043731689453125;1.218493652045292474639381907763890922069549560546875]
      mask Display: e = 0.06;c1 = [120 150 230]/255;c2 = ([120 150 230]+0)/383;c3 = ([120 150 230]+128)/383;patch([0 1 1 0],[0 0 1 1],c1);patch([0 1 1 1-e 1-e 0+e],[0 0 1 1-e 0+e 0+e],c2);patch([0 0 1 1-e 0+e 0+e],[0 1 1 1-e 1-e 0+e],c3);plot([0 1 1 0 0],[0 0 1 1 0]);disp('weights');
  "IW{2,1}(356,:)'" : Constant  Value=[0.993492037136750383297112421132624149322509765625;-0.40739188629628209081801060165162198245525360107421875;-1.0498616360300605521160832722671329975128173828125;-2.03459606632211720267378041171468794345855712890625;1.4654433294107349627921621504356153309345245361328125;0.06754436243359986102863246060223900713026523590087890625;-0.039721845193966910658733837635736563242971897125244140625;1.6410106462039995012247572958585806190967559814453125]
      mask Display: e = 0.06;c1 = [120 150 230]/255;c2 = ([120 150 230]+0)/383;c3 = ([120 150 230]+128)/383;patch([0 1 1 0],[0 0 1 1],c1);patch([0 1 1 1-e 1-e 0+e],[0 0 1 1-e 0+e 0+e],c2);patch([0 0 1 1-e 0+e 0+e],[0 1 1 1-e 1-e 0+e],c3);plot([0 1 1 0 0],[0 0 1 1 0]);disp('weights');
  "IW{2,1}(357,:)'" : Constant  Value=[1.3585612062535357136283664658549241721630096435546875;0.83124143213106116423460889564012177288532257080078125;0.59810516886082554233183827818720601499080657958984375;1.7638298969973946750400273231207393109798431396484375;1.5069564749901489530969911356805823743343353271484375;-1.375396215143826594839993049390614032745361328125;0.9907497640462619159507084987126290798187255859375;0.1225319696716461181917878775493591092526912689208984375]
      mask Display: e = 0.06;c1 = [120 150 230]/255;c2 = ([120 150 230]+0)/383;c3 = ([120 150 230]+128)/383;patch([0 1 1 0],[0 0 1 1],c1);patch([0 1 1 1-e 1-e 0+e],[0 0 1 1-e 0+e 0+e],c2);patch([0 0 1 1-e 0+e 0+e],[0 1 1 1-e 1-e 0+e],c3);plot([0 1 1 0 0],[0 0 1 1 0]);disp('weights');
  "IW{2,1}(358,:)'" : Constant  Value=[-1.4897720881707592344156410035793669521808624267578125;-1.6996479720895629750287980641587637364864349365234375;-1.11130574267857440418083569966256618499755859375;-0.6016304903270219828215203961008228361606597900390625;-0.411291933660831166008620130014605820178985595703125;-1.21527631500105126605149052920751273632049560546875;1.072393654012576025280623071012087166309356689453125;1.03316086882829072379763601929880678653717041015625]
      mask Display: e = 0.06;c1 = [120 150 230]/255;c2 = ([120 150 230]+0)/383;c3 = ([120 150 230]+128)/383;patch([0 1 1 0],[0 0 1 1],c1);patch([0 1 1 1-e 1-e 0+e],[0 0 1 1-e 0+e 0+e],c2);patch([0 0 1 1-e 0+e 0+e],[0 1 1 1-e 1-e 0+e],c3);plot([0 1 1 0 0],[0 0 1 1 0]);disp('weights');
  "IW{2,1}(359,:)'" : Constant  Value=[1.831754084721137321167816480738110840320587158203125;-0.60025053058380539727778568703797645866870880126953125;1.074288516205484711463213898241519927978515625;1.3801471533409210845633197095594368875026702880859375;-1.366983207017783197301241671084426343441009521484375;0.381661587400070889675163243737188167870044708251953125;1.187504495064237719503807966248132288455963134765625;-0.9667262455848064650609785530832596123218536376953125]
      mask Display: e = 0.06;c1 = [120 150 230]/255;c2 = ([120 150 230]+0)/383;c3 = ([120 150 230]+128)/383;patch([0 1 1 0],[0 0 1 1],c1);patch([0 1 1 1-e 1-e 0+e],[0 0 1 1-e 0+e 0+e],c2);patch([0 0 1 1-e 0+e 0+e],[0 1 1 1-e 1-e 0+e],c3);plot([0 1 1 0 0],[0 0 1 1 0]);disp('weights');
  "IW{2,1}(36,:)'" : Constant  Value=[0.870209385706692817308294252143241465091705322265625;0.64665727574552234191429533893824554979801177978515625;-0.043557528528442503168438548755148076452314853668212890625;0.67548230211788051757793027718435041606426239013671875;0.71547220555753365811568755816551856696605682373046875;1.075419953052190624731565549154765903949737548828125;-1.857860153754808951731547495000995695590972900390625;-1.9856636292778213626064598429366014897823333740234375]
      mask Display: e = 0.06;c1 = [120 150 230]/255;c2 = ([120 150 230]+0)/383;c3 = ([120 150 230]+128)/383;patch([0 1 1 0],[0 0 1 1],c1);patch([0 1 1 1-e 1-e 0+e],[0 0 1 1-e 0+e 0+e],c2);patch([0 0 1 1-e 0+e 0+e],[0 1 1 1-e 1-e 0+e],c3);plot([0 1 1 0 0],[0 0 1 1 0]);disp('weights');
  "IW{2,1}(360,:)'" : Constant  Value=[-1.45593955693627830072500728419981896877288818359375;0.12447920001931679634399330325322807766497135162353515625;-1.5134300192359215753157286599162034690380096435546875;-1.5330963721292771850812641787342727184295654296875;0.8572752717347651429946608914178796112537384033203125;0.1286170758082407494793386604214902035892009735107421875;1.8036071217805031974279472706257365643978118896484375;0.51401772221024522036003645553137175738811492919921875]
      mask Display: e = 0.06;c1 = [120 150 230]/255;c2 = ([120 150 230]+0)/383;c3 = ([120 150 230]+128)/383;patch([0 1 1 0],[0 0 1 1],c1);patch([0 1 1 1-e 1-e 0+e],[0 0 1 1-e 0+e 0+e],c2);patch([0 0 1 1-e 0+e 0+e],[0 1 1 1-e 1-e 0+e],c3);plot([0 1 1 0 0],[0 0 1 1 0]);disp('weights');
  "IW{2,1}(361,:)'" : Constant  Value=[-1.8104702706004669465755796409212052822113037109375;-1.850480422412681402732914648368023335933685302734375;-0.357577905934154338662978034335537813603878021240234375;0.83328909753239444047068218424101360142230987548828125;-0.125437809323513838055674796123639680445194244384765625;-0.9098531991427734055832843296229839324951171875;1.56696034822446250700522796250879764556884765625;-0.747489509248907335603462342987768352031707763671875]
      mask Display: e = 0.06;c1 = [120 150 230]/255;c2 = ([120 150 230]+0)/383;c3 = ([120 150 230]+128)/383;patch([0 1 1 0],[0 0 1 1],c1);patch([0 1 1 1-e 1-e 0+e],[0 0 1 1-e 0+e 0+e],c2);patch([0 0 1 1-e 0+e 0+e],[0 1 1 1-e 1-e 0+e],c3);plot([0 1 1 0 0],[0 0 1 1 0]);disp('weights');
  "IW{2,1}(362,:)'" : Constant  Value=[1.4543412599375500349196954630315303802490234375;-0.586610904293566992606656640418805181980133056640625;-0.589518599474171622887297417037189006805419921875;-1.37291537614631575792145667946897447109222412109375;-0.72657985016918846810085597098805010318756103515625;1.77110360951283940522671400685794651508331298828125;-0.80647425835136932192881431546993553638458251953125;1.60677927794890340607025791541673243045806884765625]
      mask Display: e = 0.06;c1 = [120 150 230]/255;c2 = ([120 150 230]+0)/383;c3 = ([120 150 230]+128)/383;patch([0 1 1 0],[0 0 1 1],c1);patch([0 1 1 1-e 1-e 0+e],[0 0 1 1-e 0+e 0+e],c2);patch([0 0 1 1-e 0+e 0+e],[0 1 1 1-e 1-e 0+e],c3);plot([0 1 1 0 0],[0 0 1 1 0]);disp('weights');
  "IW{2,1}(363,:)'" : Constant  Value=[1.467428385557149272955257401918061077594757080078125;0.948691041396105827487872375058941543102264404296875;0.8942204951511978361367027900996617972850799560546875;1.491800735647311082487931344076059758663177490234375;-1.5775627836035324147445635389885865151882171630859375;0.8517980333731660635976368212141096591949462890625;-1.09356057905053294376784833730198442935943603515625;-0.8498452642537481782625263804220594465732574462890625]
      mask Display: e = 0.06;c1 = [120 150 230]/255;c2 = ([120 150 230]+0)/383;c3 = ([120 150 230]+128)/383;patch([0 1 1 0],[0 0 1 1],c1);patch([0 1 1 1-e 1-e 0+e],[0 0 1 1-e 0+e 0+e],c2);patch([0 0 1 1-e 0+e 0+e],[0 1 1 1-e 1-e 0+e],c3);plot([0 1 1 0 0],[0 0 1 1 0]);disp('weights');
  "IW{2,1}(364,:)'" : Constant  Value=[-1.3690845894555414563598105814890004694461822509765625;0.96504879007393906675815742346458137035369873046875;-1.01769727396696918475527127156965434551239013671875;0.159747019669004897135522469397983513772487640380859375;-0.5276514669450367289726955277728848159313201904296875;1.671341225635934346627209379221312701702117919921875;-1.5404512273867798644033655364182777702808380126953125;-1.3857358793525691442738434489001519978046417236328125]
      mask Display: e = 0.06;c1 = [120 150 230]/255;c2 = ([120 150 230]+0)/383;c3 = ([120 150 230]+128)/383;patch([0 1 1 0],[0 0 1 1],c1);patch([0 1 1 1-e 1-e 0+e],[0 0 1 1-e 0+e 0+e],c2);patch([0 0 1 1-e 0+e 0+e],[0 1 1 1-e 1-e 0+e],c3);plot([0 1 1 0 0],[0 0 1 1 0]);disp('weights');
  "IW{2,1}(365,:)'" : Constant  Value=[1.458911527038184718918500948348082602024078369140625;-0.405601119224816120123477958259172737598419189453125;1.13320206182602856159746806952171027660369873046875;-1.0913926534113056465713498255354352295398712158203125;1.4134144731809126227517481311224400997161865234375;-0.1811262238156790271847995654752594418823719024658203125;-2.010593746838683415489867911674082279205322265625;-0.155601111342884956822985031976713798940181732177734375]
      mask Display: e = 0.06;c1 = [120 150 230]/255;c2 = ([120 150 230]+0)/383;c3 = ([120 150 230]+128)/383;patch([0 1 1 0],[0 0 1 1],c1);patch([0 1 1 1-e 1-e 0+e],[0 0 1 1-e 0+e 0+e],c2);patch([0 0 1 1-e 0+e 0+e],[0 1 1 1-e 1-e 0+e],c3);plot([0 1 1 0 0],[0 0 1 1 0]);disp('weights');
  "IW{2,1}(366,:)'" : Constant  Value=[-0.1435925935461509206358954315874143503606319427490234375;3.33028472080507643928067029737150051005301065742969512939453125e-05;1.49572842655238158471320275566540658473968505859375;-0.77766338256261768879795681641553528606891632080078125;-1.4281952818615268885338309701182879507541656494140625;0.9940534161757577091833582016988657414913177490234375;1.9148863339726691634723465540446341037750244140625;1.2176667944124177633824501754133962094783782958984375]
      mask Display: e = 0.06;c1 = [120 150 230]/255;c2 = ([120 150 230]+0)/383;c3 = ([120 150 230]+128)/383;patch([0 1 1 0],[0 0 1 1],c1);patch([0 1 1 1-e 1-e 0+e],[0 0 1 1-e 0+e 0+e],c2);patch([0 0 1 1-e 0+e 0+e],[0 1 1 1-e 1-e 0+e],c3);plot([0 1 1 0 0],[0 0 1 1 0]);disp('weights');
  "IW{2,1}(367,:)'" : Constant  Value=[1.3948825336440850986008399559068493545055389404296875;-1.0631343655614238219442313493345864117145538330078125;0.058684061090425058970776461819696123711764812469482421875;-1.31248724933893168298482123645953834056854248046875;1.112063164571190920781873501255176961421966552734375;1.567784796925779655651922439574263989925384521484375;0.4403881422533950651398981790407560765743255615234375;-1.5307272810544263474952231263159774243831634521484375]
      mask Display: e = 0.06;c1 = [120 150 230]/255;c2 = ([120 150 230]+0)/383;c3 = ([120 150 230]+128)/383;patch([0 1 1 0],[0 0 1 1],c1);patch([0 1 1 1-e 1-e 0+e],[0 0 1 1-e 0+e 0+e],c2);patch([0 0 1 1-e 0+e 0+e],[0 1 1 1-e 1-e 0+e],c3);plot([0 1 1 0 0],[0 0 1 1 0]);disp('weights');
  "IW{2,1}(368,:)'" : Constant  Value=[1.3932148808204687373546448725392110645771026611328125;1.331932229639807729881795239634811878204345703125;1.61632001693106364115237738587893545627593994140625;1.2405346254072517897526495289639569818973541259765625;-1.1086123972102057688715603944729082286357879638671875;0.601161342446035806830195724614895880222320556640625;-0.1850204350674078679350742504539084620773792266845703125;-1.1919074910233231623379879238200373947620391845703125]
      mask Display: e = 0.06;c1 = [120 150 230]/255;c2 = ([120 150 230]+0)/383;c3 = ([120 150 230]+128)/383;patch([0 1 1 0],[0 0 1 1],c1);patch([0 1 1 1-e 1-e 0+e],[0 0 1 1-e 0+e 0+e],c2);patch([0 0 1 1-e 0+e 0+e],[0 1 1 1-e 1-e 0+e],c3);plot([0 1 1 0 0],[0 0 1 1 0]);disp('weights');
  "IW{2,1}(369,:)'" : Constant  Value=[-0.55015595067380684835001147803268395364284515380859375;-2.1456516476024614092921183328144252300262451171875;-1.101881020182806647511597475386224687099456787109375;0.0130016357976382272709781062758338521234691143035888671875;-1.4816877701254338450809200367075391113758087158203125;-0.12780478952269469505864663005922921001911163330078125;-1.2517820242400661268078465582220815122127532958984375;0.9943192436589376459465938751236535608768463134765625]
      mask Display: e = 0.06;c1 = [120 150 230]/255;c2 = ([120 150 230]+0)/383;c3 = ([120 150 230]+128)/383;patch([0 1 1 0],[0 0 1 1],c1);patch([0 1 1 1-e 1-e 0+e],[0 0 1 1-e 0+e 0+e],c2);patch([0 0 1 1-e 0+e 0+e],[0 1 1 1-e 1-e 0+e],c3);plot([0 1 1 0 0],[0 0 1 1 0]);disp('weights');
  "IW{2,1}(37,:)'" : Constant  Value=[-0.6633053936199744260449051580508239567279815673828125;-1.3840420800666850542626207243301905691623687744140625;0.59111205590375026641680733519024215638637542724609375;0.3582750024304981462108798950794152915477752685546875;-0.76369450516828807362657016710727475583553314208984375;1.98682813658730150763176425243727862834930419921875;1.332883781599864203570859899627976119518280029296875;1.370287799199335410094136022962629795074462890625]
      mask Display: e = 0.06;c1 = [120 150 230]/255;c2 = ([120 150 230]+0)/383;c3 = ([120 150 230]+128)/383;patch([0 1 1 0],[0 0 1 1],c1);patch([0 1 1 1-e 1-e 0+e],[0 0 1 1-e 0+e 0+e],c2);patch([0 0 1 1-e 0+e 0+e],[0 1 1 1-e 1-e 0+e],c3);plot([0 1 1 0 0],[0 0 1 1 0]);disp('weights');
  "IW{2,1}(370,:)'" : Constant  Value=[-1.0517952201635722975225917252828367054462432861328125;-0.973625585930381731714078341610729694366455078125;0.52497560976455692749453874057508073747158050537109375;0.68702733457609943545918440577224828302860260009765625;-2.178762256737825975250189003418199717998504638671875;1.22078867193661011469885124824941158294677734375;0.0391976875310567074439660473217372782528400421142578125;-1.398928489444821732234913724823854863643646240234375]
      mask Display: e = 0.06;c1 = [120 150 230]/255;c2 = ([120 150 230]+0)/383;c3 = ([120 150 230]+128)/383;patch([0 1 1 0],[0 0 1 1],c1);patch([0 1 1 1-e 1-e 0+e],[0 0 1 1-e 0+e 0+e],c2);patch([0 0 1 1-e 0+e 0+e],[0 1 1 1-e 1-e 0+e],c3);plot([0 1 1 0 0],[0 0 1 1 0]);disp('weights');
  "IW{2,1}(371,:)'" : Constant  Value=[0.520167356604733566172171776997856795787811279296875;-1.1727653480586035517063692168449051678180694580078125;-1.2599437905808026361142992755048908293247222900390625;2.06361740277369865026457773637957870960235595703125;0.374824657590180410071667438387521542608737945556640625;1.043548325071110838280219468288123607635498046875;-0.71616528844810523057873297148034907877445220947265625;-1.3575586692239525188341531247715465724468231201171875]
      mask Display: e = 0.06;c1 = [120 150 230]/255;c2 = ([120 150 230]+0)/383;c3 = ([120 150 230]+128)/383;patch([0 1 1 0],[0 0 1 1],c1);patch([0 1 1 1-e 1-e 0+e],[0 0 1 1-e 0+e 0+e],c2);patch([0 0 1 1-e 0+e 0+e],[0 1 1 1-e 1-e 0+e],c3);plot([0 1 1 0 0],[0 0 1 1 0]);disp('weights');
  "IW{2,1}(372,:)'" : Constant  Value=[1.3269741277774584897741760869394056499004364013671875;1.500594336617201207673133467324078083038330078125;1.1721545893073341826351452255039475858211517333984375;-0.80125163275685107322487965575419366359710693359375;-1.1313551303580047235897154678241349756717681884765625;1.38227430072469470445639672107063233852386474609375;0.749564509325671313177963384077884256839752197265625;-1.0323691502564444899547879685997031629085540771484375]
      mask Display: e = 0.06;c1 = [120 150 230]/255;c2 = ([120 150 230]+0)/383;c3 = ([120 150 230]+128)/383;patch([0 1 1 0],[0 0 1 1],c1);patch([0 1 1 1-e 1-e 0+e],[0 0 1 1-e 0+e 0+e],c2);patch([0 0 1 1-e 0+e 0+e],[0 1 1 1-e 1-e 0+e],c3);plot([0 1 1 0 0],[0 0 1 1 0]);disp('weights');
  "IW{2,1}(373,:)'" : Constant  Value=[0.346507667890639858843115916897659189999103546142578125;1.466846103264405787314217377570457756519317626953125;1.5111696928799329686654573379200883209705352783203125;0.96098530684511074273501662901253439486026763916015625;0.491831931464210558857530486420728266239166259765625;-0.72554878989275117806556636423920281231403350830078125;-1.4222062910514881028944955687620677053928375244140625;1.6648749095266437425522099147201515734195709228515625]
      mask Display: e = 0.06;c1 = [120 150 230]/255;c2 = ([120 150 230]+0)/383;c3 = ([120 150 230]+128)/383;patch([0 1 1 0],[0 0 1 1],c1);patch([0 1 1 1-e 1-e 0+e],[0 0 1 1-e 0+e 0+e],c2);patch([0 0 1 1-e 0+e 0+e],[0 1 1 1-e 1-e 0+e],c3);plot([0 1 1 0 0],[0 0 1 1 0]);disp('weights');
  "IW{2,1}(374,:)'" : Constant  Value=[0.311953297913205418456783490910311229526996612548828125;1.2014860871909960327030830740113742649555206298828125;-1.650154178735764531893437379039824008941650390625;0.269100633801401645239792514985310845077037811279296875;0.32963440321797321530539193190634250640869140625;-1.1591391045858461250617210680502466857433319091796875;1.43335212657947597136853801202960312366485595703125;-1.8238919958717325631170069755171425640583038330078125]
      mask Display: e = 0.06;c1 = [120 150 230]/255;c2 = ([120 150 230]+0)/383;c3 = ([120 150 230]+128)/383;patch([0 1 1 0],[0 0 1 1],c1);patch([0 1 1 1-e 1-e 0+e],[0 0 1 1-e 0+e 0+e],c2);patch([0 0 1 1-e 0+e 0+e],[0 1 1 1-e 1-e 0+e],c3);plot([0 1 1 0 0],[0 0 1 1 0]);disp('weights');
  "IW{2,1}(375,:)'" : Constant  Value=[0.5123437862651150087600626648054458200931549072265625;1.385355486537390046208884086809121072292327880859375;1.2101402325845531660064580137259326875209808349609375;1.226528787646412599343648253125138580799102783203125;-1.5879570346842288852684532685088925063610076904296875;1.0358715522070445214097844655043445527553558349609375;-1.199304287988022910127483555697835981845855712890625;-0.95145680432471113618930758093483746051788330078125]
      mask Display: e = 0.06;c1 = [120 150 230]/255;c2 = ([120 150 230]+0)/383;c3 = ([120 150 230]+128)/383;patch([0 1 1 0],[0 0 1 1],c1);patch([0 1 1 1-e 1-e 0+e],[0 0 1 1-e 0+e 0+e],c2);patch([0 0 1 1-e 0+e 0+e],[0 1 1 1-e 1-e 0+e],c3);plot([0 1 1 0 0],[0 0 1 1 0]);disp('weights');
  "IW{2,1}(376,:)'" : Constant  Value=[0.789874567557603324274850820074789226055145263671875;0.74552950872726564401915538837783969938755035400390625;-1.4313821024496899969591368062538094818592071533203125;1.08154868700017825489112510695122182369232177734375;0.76140678796659433391624816067633219063282012939453125;1.2253114679855097168825750486575998365879058837890625;-1.1097390322151683417217782334773801267147064208984375;-1.77561177841135720001375375431962311267852783203125]
      mask Display: e = 0.06;c1 = [120 150 230]/255;c2 = ([120 150 230]+0)/383;c3 = ([120 150 230]+128)/383;patch([0 1 1 0],[0 0 1 1],c1);patch([0 1 1 1-e 1-e 0+e],[0 0 1 1-e 0+e 0+e],c2);patch([0 0 1 1-e 0+e 0+e],[0 1 1 1-e 1-e 0+e],c3);plot([0 1 1 0 0],[0 0 1 1 0]);disp('weights');
  "IW{2,1}(377,:)'" : Constant  Value=[-0.72487233700150943693785166033194400370121002197265625;1.465024616474511542918435225146822631359100341796875;0.233561364674421623188749208566150628030300140380859375;-0.1930148923448996300944457971127121709287166595458984375;-1.54679897767328355939753237180411815643310546875;1.1103079185514417304148082621395587921142578125;-1.1344606724223622595815186286927200853824615478515625;-1.80620355505280638652720881509594619274139404296875]
      mask Display: e = 0.06;c1 = [120 150 230]/255;c2 = ([120 150 230]+0)/383;c3 = ([120 150 230]+128)/383;patch([0 1 1 0],[0 0 1 1],c1);patch([0 1 1 1-e 1-e 0+e],[0 0 1 1-e 0+e 0+e],c2);patch([0 0 1 1-e 0+e 0+e],[0 1 1 1-e 1-e 0+e],c3);plot([0 1 1 0 0],[0 0 1 1 0]);disp('weights');
  "IW{2,1}(378,:)'" : Constant  Value=[-0.7769767598523318330450138091691769659519195556640625;0.299213540584596981997123066321364603936672210693359375;-0.0820452036208796087191075230293790809810161590576171875;0.425254411454966174677139179038931615650653839111328125;0.00095620419535119593502925372519030133844353258609771728515625;1.4308886936424329849870673569967038929462432861328125;2.04595742397350921493170972098596394062042236328125;1.9701850118317667526213199380435980856418609619140625]
      mask Display: e = 0.06;c1 = [120 150 230]/255;c2 = ([120 150 230]+0)/383;c3 = ([120 150 230]+128)/383;patch([0 1 1 0],[0 0 1 1],c1);patch([0 1 1 1-e 1-e 0+e],[0 0 1 1-e 0+e 0+e],c2);patch([0 0 1 1-e 0+e 0+e],[0 1 1 1-e 1-e 0+e],c3);plot([0 1 1 0 0],[0 0 1 1 0]);disp('weights');
  "IW{2,1}(379,:)'" : Constant  Value=[-1.8594094501587330459102531676762737333774566650390625;0.3203423629036386000024094755644910037517547607421875;-0.414896422047887070139182696948410011827945709228515625;-0.5512976745291624514067052587051875889301300048828125;-0.324647869925801468848902686659130267798900604248046875;-1.826299779031158809772250606329180300235748291015625;1.8213008779207384701948058136622421443462371826171875;0.407066853240525716728370753116905689239501953125]
      mask Display: e = 0.06;c1 = [120 150 230]/255;c2 = ([120 150 230]+0)/383;c3 = ([120 150 230]+128)/383;patch([0 1 1 0],[0 0 1 1],c1);patch([0 1 1 1-e 1-e 0+e],[0 0 1 1-e 0+e 0+e],c2);patch([0 0 1 1-e 0+e 0+e],[0 1 1 1-e 1-e 0+e],c3);plot([0 1 1 0 0],[0 0 1 1 0]);disp('weights');
  "IW{2,1}(38,:)'" : Constant  Value=[0.82266848149560234393362634364166297018527984619140625;-0.96686692337969903920935621499666012823581695556640625;0.9397565392968132425011162922601215541362762451171875;-0.124979841666113256071213299946975894272327423095703125;-1.8965420956822083287107716387254185974597930908203125;1.7261018994831605066764268485712818801403045654296875;-1.318622842165471542585919451084919273853302001953125;0.44074853326120899676965336766443215310573577880859375]
      mask Display: e = 0.06;c1 = [120 150 230]/255;c2 = ([120 150 230]+0)/383;c3 = ([120 150 230]+128)/383;patch([0 1 1 0],[0 0 1 1],c1);patch([0 1 1 1-e 1-e 0+e],[0 0 1 1-e 0+e 0+e],c2);patch([0 0 1 1-e 0+e 0+e],[0 1 1 1-e 1-e 0+e],c3);plot([0 1 1 0 0],[0 0 1 1 0]);disp('weights');
  "IW{2,1}(380,:)'" : Constant  Value=[-1.561005496799694025611415781895630061626434326171875;-1.93114362591357657805701819597743451595306396484375;0.6595908353355743880541695034480653703212738037109375;-1.0140367730299744142286044734646566212177276611328125;-1.11979681015146415035133031778968870639801025390625;-0.6818119799368400624217656513792462646961212158203125;1.3016242758031786319605771495844237506389617919921875;-0.3311791976975209106370812150998972356319427490234375]
      mask Display: e = 0.06;c1 = [120 150 230]/255;c2 = ([120 150 230]+0)/383;c3 = ([120 150 230]+128)/383;patch([0 1 1 0],[0 0 1 1],c1);patch([0 1 1 1-e 1-e 0+e],[0 0 1 1-e 0+e 0+e],c2);patch([0 0 1 1-e 0+e 0+e],[0 1 1 1-e 1-e 0+e],c3);plot([0 1 1 0 0],[0 0 1 1 0]);disp('weights');
  "IW{2,1}(381,:)'" : Constant  Value=[0.73223019297982860909002056359895505011081695556640625;-2.132804595376970979714315035380423069000244140625;1.2834463046455024670677858011913485825061798095703125;-1.4314802028903053088271235537831671535968780517578125;-1.1924266334316808713111868200940079987049102783203125;0.205512189265684319661176004956359975039958953857421875;0.272116135694380589793439639834105037152767181396484375;0.85475096965389518732791884758626110851764678955078125]
      mask Display: e = 0.06;c1 = [120 150 230]/255;c2 = ([120 150 230]+0)/383;c3 = ([120 150 230]+128)/383;patch([0 1 1 0],[0 0 1 1],c1);patch([0 1 1 1-e 1-e 0+e],[0 0 1 1-e 0+e 0+e],c2);patch([0 0 1 1-e 0+e 0+e],[0 1 1 1-e 1-e 0+e],c3);plot([0 1 1 0 0],[0 0 1 1 0]);disp('weights');
  "IW{2,1}(382,:)'" : Constant  Value=[1.4288755647415618543760729153291322290897369384765625;-0.383000899087571677892327670633676461875438690185546875;1.315117739034472155168487006449140608310699462890625;-1.56408551843076981668900771182961761951446533203125;0.94830115184266094985332529176957905292510986328125;1.8096904920066467781225583166815340518951416015625;-0.08462893461370703251933633737280615605413913726806640625;0.59403283295670927799392302404157817363739013671875]
      mask Display: e = 0.06;c1 = [120 150 230]/255;c2 = ([120 150 230]+0)/383;c3 = ([120 150 230]+128)/383;patch([0 1 1 0],[0 0 1 1],c1);patch([0 1 1 1-e 1-e 0+e],[0 0 1 1-e 0+e 0+e],c2);patch([0 0 1 1-e 0+e 0+e],[0 1 1 1-e 1-e 0+e],c3);plot([0 1 1 0 0],[0 0 1 1 0]);disp('weights');
  "IW{2,1}(383,:)'" : Constant  Value=[-0.0169927865260227038690654666197588085196912288665771484375;1.5498494258186863437032343426835723221302032470703125;-0.07589058922645909588400314760292530991137027740478515625;-1.4360603965411480320568671231740154325962066650390625;1.5740316227351769384767976589500904083251953125;-0.61013526506222925949174396009766496717929840087890625;-0.5514215617186872808730413453304208815097808837890625;-1.87127783209929265950677290675230324268341064453125]
      mask Display: e = 0.06;c1 = [120 150 230]/255;c2 = ([120 150 230]+0)/383;c3 = ([120 150 230]+128)/383;patch([0 1 1 0],[0 0 1 1],c1);patch([0 1 1 1-e 1-e 0+e],[0 0 1 1-e 0+e 0+e],c2);patch([0 0 1 1-e 0+e 0+e],[0 1 1 1-e 1-e 0+e],c3);plot([0 1 1 0 0],[0 0 1 1 0]);disp('weights');
  "IW{2,1}(384,:)'" : Constant  Value=[1.423252566354063386455663930973969399929046630859375;-0.131461667588464614642163041935418732464313507080078125;0.12199878340382901142913141256940434686839580535888671875;1.322011467849943056052097745123319327831268310546875;-1.6419470650177909742950532745453529059886932373046875;-1.0819860436138137860240249210619367659091949462890625;0.78865383446174863735222970717586576938629150390625;1.6019100982584910664030530824675224721431732177734375]
      mask Display: e = 0.06;c1 = [120 150 230]/255;c2 = ([120 150 230]+0)/383;c3 = ([120 150 230]+128)/383;patch([0 1 1 0],[0 0 1 1],c1);patch([0 1 1 1-e 1-e 0+e],[0 0 1 1-e 0+e 0+e],c2);patch([0 0 1 1-e 0+e 0+e],[0 1 1 1-e 1-e 0+e],c3);plot([0 1 1 0 0],[0 0 1 1 0]);disp('weights');
  "IW{2,1}(385,:)'" : Constant  Value=[1.1462188115797167231590947267250157892704010009765625;-1.271752144115979366034707709331996738910675048828125;1.200674761614294538958347402513027191162109375;1.1725153346890631045340569471591152250766754150390625;1.537186567624220234762333348044194281101226806640625;1.519161877666797000330234368448145687580108642578125;0.038006466050880725882077371124978526495397090911865234375;-0.74192600403363062611106215626932680606842041015625]
      mask Display: e = 0.06;c1 = [120 150 230]/255;c2 = ([120 150 230]+0)/383;c3 = ([120 150 230]+128)/383;patch([0 1 1 0],[0 0 1 1],c1);patch([0 1 1 1-e 1-e 0+e],[0 0 1 1-e 0+e 0+e],c2);patch([0 0 1 1-e 0+e 0+e],[0 1 1 1-e 1-e 0+e],c3);plot([0 1 1 0 0],[0 0 1 1 0]);disp('weights');
  "IW{2,1}(386,:)'" : Constant  Value=[-0.88572956092145982420760219611111097037792205810546875;1.93570701704177583479804525268264114856719970703125;-0.32262167638336125552456223886110819876194000244140625;0.92872999621708929307573043843149207532405853271484375;0.8688996541955400498835615508141927421092987060546875;0.1686611154557091374339705680540646426379680633544921875;-1.460492212527837008195774615160189568996429443359375;-1.697037784030266838186662425869144499301910400390625]
      mask Display: e = 0.06;c1 = [120 150 230]/255;c2 = ([120 150 230]+0)/383;c3 = ([120 150 230]+128)/383;patch([0 1 1 0],[0 0 1 1],c1);patch([0 1 1 1-e 1-e 0+e],[0 0 1 1-e 0+e 0+e],c2);patch([0 0 1 1-e 0+e 0+e],[0 1 1 1-e 1-e 0+e],c3);plot([0 1 1 0 0],[0 0 1 1 0]);disp('weights');
  "IW{2,1}(387,:)'" : Constant  Value=[-0.47150987099022667603520631018909625709056854248046875;0.9559304672859865181777649922878481447696685791015625;1.987779374731089898631353207747451961040496826171875;0.358418598563045254223879965138621628284454345703125;-0.81808486629852461557987908236100338399410247802734375;-1.353187842197297374724485052865929901599884033203125;-1.0559832404559872376381690628477372229099273681640625;1.5613416107838593571699448148137889802455902099609375]
      mask Display: e = 0.06;c1 = [120 150 230]/255;c2 = ([120 150 230]+0)/383;c3 = ([120 150 230]+128)/383;patch([0 1 1 0],[0 0 1 1],c1);patch([0 1 1 1-e 1-e 0+e],[0 0 1 1-e 0+e 0+e],c2);patch([0 0 1 1-e 0+e 0+e],[0 1 1 1-e 1-e 0+e],c3);plot([0 1 1 0 0],[0 0 1 1 0]);disp('weights');
  "IW{2,1}(388,:)'" : Constant  Value=[-0.051348282467908734627570765951531939208507537841796875;-2.23173585870506929751400093664415180683135986328125;-0.6665365932699971462938037802814505994319915771484375;-0.1589141118214207060166387464050785638391971588134765625;-0.386169785643835583588412418976076878607273101806640625;0.175694404558804750937639482799568213522434234619140625;0.268398202820408549040820389564032666385173797607421875;-2.24881191335504748707307953736744821071624755859375]
      mask Display: e = 0.06;c1 = [120 150 230]/255;c2 = ([120 150 230]+0)/383;c3 = ([120 150 230]+128)/383;patch([0 1 1 0],[0 0 1 1],c1);patch([0 1 1 1-e 1-e 0+e],[0 0 1 1-e 0+e 0+e],c2);patch([0 0 1 1-e 0+e 0+e],[0 1 1 1-e 1-e 0+e],c3);plot([0 1 1 0 0],[0 0 1 1 0]);disp('weights');
  "IW{2,1}(389,:)'" : Constant  Value=[-1.8020655856834582042580450433888472616672515869140625;-0.7384412267140529895215195210766978561878204345703125;0.75584713158981997604968228188226930797100067138671875;-1.599538232441755081225664980593137443065643310546875;-0.2297839401018963167988573559341602958738803863525390625;-0.74999440976091680255422033951617777347564697265625;-1.8289632468998819891936591375269927084445953369140625;-0.345199751620103689742080632640863768756389617919921875]
      mask Display: e = 0.06;c1 = [120 150 230]/255;c2 = ([120 150 230]+0)/383;c3 = ([120 150 230]+128)/383;patch([0 1 1 0],[0 0 1 1],c1);patch([0 1 1 1-e 1-e 0+e],[0 0 1 1-e 0+e 0+e],c2);patch([0 0 1 1-e 0+e 0+e],[0 1 1 1-e 1-e 0+e],c3);plot([0 1 1 0 0],[0 0 1 1 0]);disp('weights');
  "IW{2,1}(39,:)'" : Constant  Value=[-0.060735793655545246283455895763836451806128025054931640625;0.71308237757141113011272182120592333376407623291015625;0.61114972233778608323717662642593495547771453857421875;1.513188087227655298505624159588478505611419677734375;1.378461003453590905110104358755052089691162109375;-1.4626444447395787751275975097087211906909942626953125;1.204662798197551953904849142418242990970611572265625;1.535946093080053032053911010734736919403076171875]
      mask Display: e = 0.06;c1 = [120 150 230]/255;c2 = ([120 150 230]+0)/383;c3 = ([120 150 230]+128)/383;patch([0 1 1 0],[0 0 1 1],c1);patch([0 1 1 1-e 1-e 0+e],[0 0 1 1-e 0+e 0+e],c2);patch([0 0 1 1-e 0+e 0+e],[0 1 1 1-e 1-e 0+e],c3);plot([0 1 1 0 0],[0 0 1 1 0]);disp('weights');
  "IW{2,1}(390,:)'" : Constant  Value=[-0.50857338073543478795812688986188732087612152099609375;-0.730242759364909677088917305809445679187774658203125;0.56617537803169304400086048190132714807987213134765625;-0.63989524081910698072306331596337258815765380859375;-1.309258480446237715710822158143855631351470947265625;-2.3414793017349051496012179995886981487274169921875;-0.4815273078874102719026950580882839858531951904296875;-1.5247831694799216517566264883498661220073699951171875]
      mask Display: e = 0.06;c1 = [120 150 230]/255;c2 = ([120 150 230]+0)/383;c3 = ([120 150 230]+128)/383;patch([0 1 1 0],[0 0 1 1],c1);patch([0 1 1 1-e 1-e 0+e],[0 0 1 1-e 0+e 0+e],c2);patch([0 0 1 1-e 0+e 0+e],[0 1 1 1-e 1-e 0+e],c3);plot([0 1 1 0 0],[0 0 1 1 0]);disp('weights');
  "IW{2,1}(391,:)'" : Constant  Value=[1.5960024669897079352409718921990133821964263916015625;-1.04724741507534968576464962097816169261932373046875;0.78232287719150905846987598124542273581027984619140625;1.5091614164935671649203641209169290959835052490234375;-1.1836986251749366250152206703205592930316925048828125;0.444898172882107922898597962557687424123287200927734375;-1.3665536477761375255823850238812156021595001220703125;-1.0282900408247375168002690770663321018218994140625]
      mask Display: e = 0.06;c1 = [120 150 230]/255;c2 = ([120 150 230]+0)/383;c3 = ([120 150 230]+128)/383;patch([0 1 1 0],[0 0 1 1],c1);patch([0 1 1 1-e 1-e 0+e],[0 0 1 1-e 0+e 0+e],c2);patch([0 0 1 1-e 0+e 0+e],[0 1 1 1-e 1-e 0+e],c3);plot([0 1 1 0 0],[0 0 1 1 0]);disp('weights');
  "IW{2,1}(392,:)'" : Constant  Value=[0.312318245259008919756382738341926597058773040771484375;1.374682960101908602013054405688308179378509521484375;-2.0704241036289250388335858588106930255889892578125;-0.987669629305553353759705714765004813671112060546875;-1.80960520538502489529264494194649159908294677734375;0.276294730171518232442195994735811837017536163330078125;0.1793971254105704293824175010740873403847217559814453125;0.60506446799526603097518773211049847304821014404296875]
      mask Display: e = 0.06;c1 = [120 150 230]/255;c2 = ([120 150 230]+0)/383;c3 = ([120 150 230]+128)/383;patch([0 1 1 0],[0 0 1 1],c1);patch([0 1 1 1-e 1-e 0+e],[0 0 1 1-e 0+e 0+e],c2);patch([0 0 1 1-e 0+e 0+e],[0 1 1 1-e 1-e 0+e],c3);plot([0 1 1 0 0],[0 0 1 1 0]);disp('weights');
  "IW{2,1}(393,:)'" : Constant  Value=[0.01176744952491269070871116042553694569505751132965087890625;1.41777247110751591918642589007504284381866455078125;1.4943075379396386637154137133620679378509521484375;1.422479326161463664135453655035234987735748291015625;0.256780486608617131150111845272476784884929656982421875;-1.2892477163331452771899421350099146366119384765625;0.6062417095357985896697528005461208522319793701171875;-1.646741739354639744163932846277020871639251708984375]
      mask Display: e = 0.06;c1 = [120 150 230]/255;c2 = ([120 150 230]+0)/383;c3 = ([120 150 230]+128)/383;patch([0 1 1 0],[0 0 1 1],c1);patch([0 1 1 1-e 1-e 0+e],[0 0 1 1-e 0+e 0+e],c2);patch([0 0 1 1-e 0+e 0+e],[0 1 1 1-e 1-e 0+e],c3);plot([0 1 1 0 0],[0 0 1 1 0]);disp('weights');
  "IW{2,1}(394,:)'" : Constant  Value=[1.514055285272761341985869876225478947162628173828125;-1.555221867603970853366490700864233076572418212890625;-0.95274562029909370952651670449995435774326324462890625;0.68482057260683470989448551335954107344150543212890625;-1.6475391911709904579907970401109196245670318603515625;-1.4286468307915487496728701444226317107677459716796875;-0.18604923916827920127303741537616588175296783447265625;-0.389644909376670900424954879781580530107021331787109375]
      mask Display: e = 0.06;c1 = [120 150 230]/255;c2 = ([120 150 230]+0)/383;c3 = ([120 150 230]+128)/383;patch([0 1 1 0],[0 0 1 1],c1);patch([0 1 1 1-e 1-e 0+e],[0 0 1 1-e 0+e 0+e],c2);patch([0 0 1 1-e 0+e 0+e],[0 1 1 1-e 1-e 0+e],c3);plot([0 1 1 0 0],[0 0 1 1 0]);disp('weights');
  "IW{2,1}(395,:)'" : Constant  Value=[1.67727088470826490862464197562076151371002197265625;0.2471125593640040307708005684617091901600360870361328125;-1.524219727650850675360061359242536127567291259765625;2.166266598463186365819410639232955873012542724609375;0.65010919222282070872864778721123002469539642333984375;0.62835998849042429270639331662096083164215087890625;-0.07881816327904832275574875666279694996774196624755859375;-0.494977450626986115178596037367242388427257537841796875]
      mask Display: e = 0.06;c1 = [120 150 230]/255;c2 = ([120 150 230]+0)/383;c3 = ([120 150 230]+128)/383;patch([0 1 1 0],[0 0 1 1],c1);patch([0 1 1 1-e 1-e 0+e],[0 0 1 1-e 0+e 0+e],c2);patch([0 0 1 1-e 0+e 0+e],[0 1 1 1-e 1-e 0+e],c3);plot([0 1 1 0 0],[0 0 1 1 0]);disp('weights');
  "IW{2,1}(396,:)'" : Constant  Value=[-0.61365923022664758956778996434877626597881317138671875;-1.7326284030884535614092101241112686693668365478515625;-0.58266368475777319257957742593134753406047821044921875;-1.166720981773554655092084431089460849761962890625;0.67313163737284342769129352745949290692806243896484375;-0.8433545033252458633654669029056094586849212646484375;-2.09641009626221741513063534512184560298919677734375;-0.647937841647582946080774490837939083576202392578125]
      mask Display: e = 0.06;c1 = [120 150 230]/255;c2 = ([120 150 230]+0)/383;c3 = ([120 150 230]+128)/383;patch([0 1 1 0],[0 0 1 1],c1);patch([0 1 1 1-e 1-e 0+e],[0 0 1 1-e 0+e 0+e],c2);patch([0 0 1 1-e 0+e 0+e],[0 1 1 1-e 1-e 0+e],c3);plot([0 1 1 0 0],[0 0 1 1 0]);disp('weights');
  "IW{2,1}(397,:)'" : Constant  Value=[-0.5752257943190282052370321252965368330478668212890625;0.88786225427388287823049495273153297603130340576171875;1.6811682932199853990340443488094024360179901123046875;-1.3566514782461249755129983896040357649326324462890625;0.589266708578936704299167104181833565235137939453125;1.06300309499220357878357390291057527065277099609375;0.15516033169644938283227020292542874813079833984375;1.9407651966296841639092463083215989172458648681640625]
      mask Display: e = 0.06;c1 = [120 150 230]/255;c2 = ([120 150 230]+0)/383;c3 = ([120 150 230]+128)/383;patch([0 1 1 0],[0 0 1 1],c1);patch([0 1 1 1-e 1-e 0+e],[0 0 1 1-e 0+e 0+e],c2);patch([0 0 1 1-e 0+e 0+e],[0 1 1 1-e 1-e 0+e],c3);plot([0 1 1 0 0],[0 0 1 1 0]);disp('weights');
  "IW{2,1}(398,:)'" : Constant  Value=[-0.64260597713009526277261329596512950956821441650390625;1.985168159489295813813214408583007752895355224609375;-0.90331042723594590082569766309461556375026702880859375;-0.55056864764715651716642241808585822582244873046875;-0.59519704134902451375666032618028111755847930908203125;0.6796861057105363368435746451723389327526092529296875;-1.687485236094091956005058818846009671688079833984375;-1.3020269372020092379926836656522937119007110595703125]
      mask Display: e = 0.06;c1 = [120 150 230]/255;c2 = ([120 150 230]+0)/383;c3 = ([120 150 230]+128)/383;patch([0 1 1 0],[0 0 1 1],c1);patch([0 1 1 1-e 1-e 0+e],[0 0 1 1-e 0+e 0+e],c2);patch([0 0 1 1-e 0+e 0+e],[0 1 1 1-e 1-e 0+e],c3);plot([0 1 1 0 0],[0 0 1 1 0]);disp('weights');
  "IW{2,1}(399,:)'" : Constant  Value=[1.2560096796672450825127498319488950073719024658203125;1.7304682535164166434782373471534810960292816162109375;-1.1711090802633974394808547003776766359806060791015625;1.191346471489356684259064422803930938243865966796875;-1.50409084672401771598515551886521279811859130859375;0.1358343552780567342619377768642152659595012664794921875;0.453747121664005492736038149814703501760959625244140625;-1.1394072403572168550311971557675860822200775146484375]
      mask Display: e = 0.06;c1 = [120 150 230]/255;c2 = ([120 150 230]+0)/383;c3 = ([120 150 230]+128)/383;patch([0 1 1 0],[0 0 1 1],c1);patch([0 1 1 1-e 1-e 0+e],[0 0 1 1-e 0+e 0+e],c2);patch([0 0 1 1-e 0+e 0+e],[0 1 1 1-e 1-e 0+e],c3);plot([0 1 1 0 0],[0 0 1 1 0]);disp('weights');
  "IW{2,1}(4,:)'" : Constant  Value=[-1.6722175142280708559638924270984716713428497314453125;-0.6186093312120071185944425451452843844890594482421875;0.41710280665912768949254996186937205493450164794921875;-1.6245343353685941512054569102474488317966461181640625;-0.93495019273919377500448035789304412901401519775390625;-1.3360554090231229196206186315976083278656005859375;0.4040986418530494450607193357427604496479034423828125;-1.474062053830223373296348654548637568950653076171875]
      mask Display: e = 0.06;c1 = [120 150 230]/255;c2 = ([120 150 230]+0)/383;c3 = ([120 150 230]+128)/383;patch([0 1 1 0],[0 0 1 1],c1);patch([0 1 1 1-e 1-e 0+e],[0 0 1 1-e 0+e 0+e],c2);patch([0 0 1 1-e 0+e 0+e],[0 1 1 1-e 1-e 0+e],c3);plot([0 1 1 0 0],[0 0 1 1 0]);disp('weights');
  "IW{2,1}(40,:)'" : Constant  Value=[1.683172212169874892850884862127713859081268310546875;1.36477193143281017029266877216286957263946533203125;-0.86026880900184188316615063740755431354045867919921875;0.807993974978623352711792904301546514034271240234375;-1.11210637915222232408041236340068280696868896484375;-0.72579849657315076427721578511409461498260498046875;-0.63209908104897050140635883508366532623767852783203125;1.703541106729399512431655239197425544261932373046875]
      mask Display: e = 0.06;c1 = [120 150 230]/255;c2 = ([120 150 230]+0)/383;c3 = ([120 150 230]+128)/383;patch([0 1 1 0],[0 0 1 1],c1);patch([0 1 1 1-e 1-e 0+e],[0 0 1 1-e 0+e 0+e],c2);patch([0 0 1 1-e 0+e 0+e],[0 1 1 1-e 1-e 0+e],c3);plot([0 1 1 0 0],[0 0 1 1 0]);disp('weights');
  "IW{2,1}(400,:)'" : Constant  Value=[-1.4211895821145763552095786508289165794849395751953125;-1.2377008548650270114421800826676189899444580078125;-1.4806660148030748036518389199045486748218536376953125;-0.05405324393545672678751401463159709237515926361083984375;0.4410436222661500149655466884723864495754241943359375;0.396960446679740786013468323289998807013034820556640625;-1.3878448270407692799466303767985664308071136474609375;-1.726533291132835490344632489723153412342071533203125]
      mask Display: e = 0.06;c1 = [120 150 230]/255;c2 = ([120 150 230]+0)/383;c3 = ([120 150 230]+128)/383;patch([0 1 1 0],[0 0 1 1],c1);patch([0 1 1 1-e 1-e 0+e],[0 0 1 1-e 0+e 0+e],c2);patch([0 0 1 1-e 0+e 0+e],[0 1 1 1-e 1-e 0+e],c3);plot([0 1 1 0 0],[0 0 1 1 0]);disp('weights');
  "IW{2,1}(401,:)'" : Constant  Value=[-0.05804372230679859245849883109258371405303478240966796875;0.65670524464667934250172720567206852138042449951171875;-1.9576770843753499296013842467800714075565338134765625;0.691432806207506356344083542353473603725433349609375;1.02938901029098683892470944556407630443572998046875;1.24914251350571792187338360236026346683502197265625;1.2066767223488252813723420331371016800403594970703125;-1.4976606857135610351150489805149845778942108154296875]
      mask Display: e = 0.06;c1 = [120 150 230]/255;c2 = ([120 150 230]+0)/383;c3 = ([120 150 230]+128)/383;patch([0 1 1 0],[0 0 1 1],c1);patch([0 1 1 1-e 1-e 0+e],[0 0 1 1-e 0+e 0+e],c2);patch([0 0 1 1-e 0+e 0+e],[0 1 1 1-e 1-e 0+e],c3);plot([0 1 1 0 0],[0 0 1 1 0]);disp('weights');
  "IW{2,1}(402,:)'" : Constant  Value=[1.4246388868916657344243503757752478122711181640625;0.201985788662728260600687235637451522052288055419921875;-1.651090993503679715814769224380142986774444580078125;1.28392554119323509809191818931140005588531494140625;-0.6406258099650383730505609491956420242786407470703125;1.5490145109822239799512999525177292525768280029296875;-1.3474695789127173473076481968746520578861236572265625;-0.706638236301818434270671787089668214321136474609375]
      mask Display: e = 0.06;c1 = [120 150 230]/255;c2 = ([120 150 230]+0)/383;c3 = ([120 150 230]+128)/383;patch([0 1 1 0],[0 0 1 1],c1);patch([0 1 1 1-e 1-e 0+e],[0 0 1 1-e 0+e 0+e],c2);patch([0 0 1 1-e 0+e 0+e],[0 1 1 1-e 1-e 0+e],c3);plot([0 1 1 0 0],[0 0 1 1 0]);disp('weights');
  "IW{2,1}(403,:)'" : Constant  Value=[0.352633096517707189665458145100274123251438140869140625;1.1483610898607725658848721650429069995880126953125;-0.7599035068595210162811781628988683223724365234375;1.3023608641774255811895955048385076224803924560546875;-0.99559979010347643413325613437336869537830352783203125;-0.85768690923286683425175169759313575923442840576171875;1.6424265110684732604795499355532228946685791015625;1.695762211638823568904399508028291165828704833984375]
      mask Display: e = 0.06;c1 = [120 150 230]/255;c2 = ([120 150 230]+0)/383;c3 = ([120 150 230]+128)/383;patch([0 1 1 0],[0 0 1 1],c1);patch([0 1 1 1-e 1-e 0+e],[0 0 1 1-e 0+e 0+e],c2);patch([0 0 1 1-e 0+e 0+e],[0 1 1 1-e 1-e 0+e],c3);plot([0 1 1 0 0],[0 0 1 1 0]);disp('weights');
  "IW{2,1}(404,:)'" : Constant  Value=[0.88610595123896629399240509883384220302104949951171875;0.69675783343007846593053500328096561133861541748046875;1.3541360646494400299388871644623577594757080078125;-0.78033178311983253383488090548780746757984161376953125;-1.5080240861019220677263774632592685520648956298828125;1.2225155717284901246699746479862369596958160400390625;-1.4342990344829276150306895942776463925838470458984375;-1.2712772855439997687909681189921684563159942626953125]
      mask Display: e = 0.06;c1 = [120 150 230]/255;c2 = ([120 150 230]+0)/383;c3 = ([120 150 230]+128)/383;patch([0 1 1 0],[0 0 1 1],c1);patch([0 1 1 1-e 1-e 0+e],[0 0 1 1-e 0+e 0+e],c2);patch([0 0 1 1-e 0+e 0+e],[0 1 1 1-e 1-e 0+e],c3);plot([0 1 1 0 0],[0 0 1 1 0]);disp('weights');
  "IW{2,1}(405,:)'" : Constant  Value=[-1.4560681621660889195624122294248081743717193603515625;-0.45847234214192644774499285631463862955570220947265625;0.52177791051456334781022405877592973411083221435546875;-1.2035276014757474438710005415487103164196014404296875;2.024107843561743447224898773129098117351531982421875;-0.279583843681671939673805127313244156539440155029296875;-1.13898086585398772285770974121987819671630859375;1.2029847306243015570004217806854285299777984619140625]
      mask Display: e = 0.06;c1 = [120 150 230]/255;c2 = ([120 150 230]+0)/383;c3 = ([120 150 230]+128)/383;patch([0 1 1 0],[0 0 1 1],c1);patch([0 1 1 1-e 1-e 0+e],[0 0 1 1-e 0+e 0+e],c2);patch([0 0 1 1-e 0+e 0+e],[0 1 1 1-e 1-e 0+e],c3);plot([0 1 1 0 0],[0 0 1 1 0]);disp('weights');
  "IW{2,1}(406,:)'" : Constant  Value=[-2.129395418256651684174585170694626867771148681640625;-1.4609796862187323096549107503960840404033660888671875;0.95711688623071300430211749699083156883716583251953125;0.490888965300289303872460777711239643394947052001953125;-0.81740338352538299826477441456518135964870452880859375;0.78955525763793843463389521275530569255352020263671875;-0.465846749897496026360244059105752967298030853271484375;1.324958496562208321023490498191677033901214599609375]
      mask Display: e = 0.06;c1 = [120 150 230]/255;c2 = ([120 150 230]+0)/383;c3 = ([120 150 230]+128)/383;patch([0 1 1 0],[0 0 1 1],c1);patch([0 1 1 1-e 1-e 0+e],[0 0 1 1-e 0+e 0+e],c2);patch([0 0 1 1-e 0+e 0+e],[0 1 1 1-e 1-e 0+e],c3);plot([0 1 1 0 0],[0 0 1 1 0]);disp('weights');
  "IW{2,1}(407,:)'" : Constant  Value=[0.45052523941102207150066760732443071901798248291015625;1.7975209835726138063449752735323272645473480224609375;-1.172409660735327374680991852073930203914642333984375;-1.258930921725625484697275169310159981250762939453125;1.6977247050527648486450971176964230835437774658203125;-0.554484387517978571935373111045919358730316162109375;-0.53503995116562308442809126063366420567035675048828125;-1.24751785351357735720512209809385240077972412109375]
      mask Display: e = 0.06;c1 = [120 150 230]/255;c2 = ([120 150 230]+0)/383;c3 = ([120 150 230]+128)/383;patch([0 1 1 0],[0 0 1 1],c1);patch([0 1 1 1-e 1-e 0+e],[0 0 1 1-e 0+e 0+e],c2);patch([0 0 1 1-e 0+e 0+e],[0 1 1 1-e 1-e 0+e],c3);plot([0 1 1 0 0],[0 0 1 1 0]);disp('weights');
  "IW{2,1}(408,:)'" : Constant  Value=[1.9462720988169459612748823928995989263057708740234375;-0.71799547254951623376229008499649353325366973876953125;0.497053937610322404960783160277060233056545257568359375;-0.66894249584568743483004027439164929091930389404296875;-1.1746208883879785123127703627687878906726837158203125;-0.68924542807268107669216306021553464233875274658203125;-1.1437931815064847906882050665444694459438323974609375;-1.7015721486356543135087804330396465957164764404296875]
      mask Display: e = 0.06;c1 = [120 150 230]/255;c2 = ([120 150 230]+0)/383;c3 = ([120 150 230]+128)/383;patch([0 1 1 0],[0 0 1 1],c1);patch([0 1 1 1-e 1-e 0+e],[0 0 1 1-e 0+e 0+e],c2);patch([0 0 1 1-e 0+e 0+e],[0 1 1 1-e 1-e 0+e],c3);plot([0 1 1 0 0],[0 0 1 1 0]);disp('weights');
  "IW{2,1}(409,:)'" : Constant  Value=[0.66405211502234051668125403011799789965152740478515625;0.39773767378580970888179990652133710682392120361328125;1.4503472321077415241319386041141115128993988037109375;-0.021015190818788408166906123142325668595731258392333984375;-1.74366416415162550634931903914548456668853759765625;1.7959137617364946404308057026355527341365814208984375;1.1409145804216345165826851371093653142452239990234375;0.8438876746302634845875445535057224333286285400390625]
      mask Display: e = 0.06;c1 = [120 150 230]/255;c2 = ([120 150 230]+0)/383;c3 = ([120 150 230]+128)/383;patch([0 1 1 0],[0 0 1 1],c1);patch([0 1 1 1-e 1-e 0+e],[0 0 1 1-e 0+e 0+e],c2);patch([0 0 1 1-e 0+e 0+e],[0 1 1 1-e 1-e 0+e],c3);plot([0 1 1 0 0],[0 0 1 1 0]);disp('weights');
  "IW{2,1}(41,:)'" : Constant  Value=[-1.2363941583632007681359255002462305128574371337890625;-1.1536338626269875273777643087669275701045989990234375;0.804884403130089243205702587147243320941925048828125;1.4108717651518019042811147301108576357364654541015625;-1.1446182592775049347011417921748943626880645751953125;-1.053878463310180979561891945195384323596954345703125;0.0416549466233120668778866502179880626499652862548828125;1.7009926270323385555371942245983518660068511962890625]
      mask Display: e = 0.06;c1 = [120 150 230]/255;c2 = ([120 150 230]+0)/383;c3 = ([120 150 230]+128)/383;patch([0 1 1 0],[0 0 1 1],c1);patch([0 1 1 1-e 1-e 0+e],[0 0 1 1-e 0+e 0+e],c2);patch([0 0 1 1-e 0+e 0+e],[0 1 1 1-e 1-e 0+e],c3);plot([0 1 1 0 0],[0 0 1 1 0]);disp('weights');
  "IW{2,1}(410,:)'" : Constant  Value=[-1.7350110896881896227483821348869241774082183837890625;-0.320125564013618191250287736693280749022960662841796875;1.743804543823582520190029754303395748138427734375;0.371264536452023008461509334665606729686260223388671875;0.5409810339139300428001888576545752584934234619140625;0.07682092214914736094666380950002348981797695159912109375;0.82243621769879193816876750133815221488475799560546875;1.9102427655000819850528159804525785148143768310546875]
      mask Display: e = 0.06;c1 = [120 150 230]/255;c2 = ([120 150 230]+0)/383;c3 = ([120 150 230]+128)/383;patch([0 1 1 0],[0 0 1 1],c1);patch([0 1 1 1-e 1-e 0+e],[0 0 1 1-e 0+e 0+e],c2);patch([0 0 1 1-e 0+e 0+e],[0 1 1 1-e 1-e 0+e],c3);plot([0 1 1 0 0],[0 0 1 1 0]);disp('weights');
  "IW{2,1}(411,:)'" : Constant  Value=[0.11670550221047680528041468051014817319810390472412109375;-1.17747570343543639381778120878152549266815185546875;1.5839901760883974279892072445363737642765045166015625;1.8542569374224218137214847956784069538116455078125;1.5267950140004182824071676805033348500728607177734375;-0.96716410401806240937361280884942971169948577880859375;0.328090082344845990203197061418904922902584075927734375;0.60574091345020086851747009859536774456501007080078125]
      mask Display: e = 0.06;c1 = [120 150 230]/255;c2 = ([120 150 230]+0)/383;c3 = ([120 150 230]+128)/383;patch([0 1 1 0],[0 0 1 1],c1);patch([0 1 1 1-e 1-e 0+e],[0 0 1 1-e 0+e 0+e],c2);patch([0 0 1 1-e 0+e 0+e],[0 1 1 1-e 1-e 0+e],c3);plot([0 1 1 0 0],[0 0 1 1 0]);disp('weights');
  "IW{2,1}(412,:)'" : Constant  Value=[-1.5060962186092818893001776814344339072704315185546875;-1.392273995373853434642796855769120156764984130859375;1.3212002297519085391996895850752480328083038330078125;-0.07076238468411977233785137286758981645107269287109375;1.2373191881076357478974614423350431025028228759765625;-0.81819745303947566394953128110500983893871307373046875;-0.00991404260786439735231301284557048347778618335723876953125;-1.6608846730895105991976379300467669963836669921875]
      mask Display: e = 0.06;c1 = [120 150 230]/255;c2 = ([120 150 230]+0)/383;c3 = ([120 150 230]+128)/383;patch([0 1 1 0],[0 0 1 1],c1);patch([0 1 1 1-e 1-e 0+e],[0 0 1 1-e 0+e 0+e],c2);patch([0 0 1 1-e 0+e 0+e],[0 1 1 1-e 1-e 0+e],c3);plot([0 1 1 0 0],[0 0 1 1 0]);disp('weights');
  "IW{2,1}(413,:)'" : Constant  Value=[0.5318621669993055522951408420340158045291900634765625;0.81733069421123027975539798717363737523555755615234375;0.582345539693417180160395218990743160247802734375;-1.7154473982671738507832515097106806933879852294921875;-0.2109965485423775100048970898569677956402301788330078125;1.509946247855237455581800531945191323757171630859375;2.099490655410200634634065863792784512042999267578125;-0.235769407656085672186918600345961749553680419921875]
      mask Display: e = 0.06;c1 = [120 150 230]/255;c2 = ([120 150 230]+0)/383;c3 = ([120 150 230]+128)/383;patch([0 1 1 0],[0 0 1 1],c1);patch([0 1 1 1-e 1-e 0+e],[0 0 1 1-e 0+e 0+e],c2);patch([0 0 1 1-e 0+e 0+e],[0 1 1 1-e 1-e 0+e],c3);plot([0 1 1 0 0],[0 0 1 1 0]);disp('weights');
  "IW{2,1}(414,:)'" : Constant  Value=[-0.236327409396584309231315046417876146733760833740234375;1.868997288749196794555018641403876245021820068359375;1.364181010798462434507882790057919919490814208984375;0.678625061830103515347900611232034862041473388671875;0.8340363337922871433960381182259880006313323974609375;-1.1587692884388030023501414689235389232635498046875;-1.7423445842588609622225703787989914417266845703125;0.08285025815994585818291540135760442353785037994384765625]
      mask Display: e = 0.06;c1 = [120 150 230]/255;c2 = ([120 150 230]+0)/383;c3 = ([120 150 230]+128)/383;patch([0 1 1 0],[0 0 1 1],c1);patch([0 1 1 1-e 1-e 0+e],[0 0 1 1-e 0+e 0+e],c2);patch([0 0 1 1-e 0+e 0+e],[0 1 1 1-e 1-e 0+e],c3);plot([0 1 1 0 0],[0 0 1 1 0]);disp('weights');
  "IW{2,1}(415,:)'" : Constant  Value=[0.9476823038714845548469156710780225694179534912109375;0.7276314091136326656084065689356066286563873291015625;1.63488631970240927415716214454732835292816162109375;0.40409390224718466644304726287373341619968414306640625;-0.88928238127793612921578869645600207149982452392578125;1.6828175952600668008329876101925037801265716552734375;-1.450914397266200861480456296703778207302093505859375;-0.9476347445016479742463388902251608669757843017578125]
      mask Display: e = 0.06;c1 = [120 150 230]/255;c2 = ([120 150 230]+0)/383;c3 = ([120 150 230]+128)/383;patch([0 1 1 0],[0 0 1 1],c1);patch([0 1 1 1-e 1-e 0+e],[0 0 1 1-e 0+e 0+e],c2);patch([0 0 1 1-e 0+e 0+e],[0 1 1 1-e 1-e 0+e],c3);plot([0 1 1 0 0],[0 0 1 1 0]);disp('weights');
  "IW{2,1}(416,:)'" : Constant  Value=[-1.7204145598898963331890854533412493765354156494140625;1.2109719883521676830895330567727796733379364013671875;1.506179106804423906140755207161419093608856201171875;0.1880986016537455618458096751055563800036907196044921875;-1.436380503994367341391580339404754340648651123046875;0.0874480931751879519975290122602018527686595916748046875;1.5653201095912183671288175901281647384166717529296875;0.0367740582307442831488941692441585473716259002685546875]
      mask Display: e = 0.06;c1 = [120 150 230]/255;c2 = ([120 150 230]+0)/383;c3 = ([120 150 230]+128)/383;patch([0 1 1 0],[0 0 1 1],c1);patch([0 1 1 1-e 1-e 0+e],[0 0 1 1-e 0+e 0+e],c2);patch([0 0 1 1-e 0+e 0+e],[0 1 1 1-e 1-e 0+e],c3);plot([0 1 1 0 0],[0 0 1 1 0]);disp('weights');
  "IW{2,1}(417,:)'" : Constant  Value=[-1.3499177232820243066413468113751150667667388916015625;-1.347739625055480505722016459912993013858795166015625;-0.332119510812249274511742669346858747303485870361328125;-1.3109353636036680246235164304380305111408233642578125;0.1995004291680057828539673892009886913001537322998046875;0.6339792961165731099981712759472429752349853515625;2.1127436406938375768049809266813099384307861328125;-0.9280871684107150354492432597908191382884979248046875]
      mask Display: e = 0.06;c1 = [120 150 230]/255;c2 = ([120 150 230]+0)/383;c3 = ([120 150 230]+128)/383;patch([0 1 1 0],[0 0 1 1],c1);patch([0 1 1 1-e 1-e 0+e],[0 0 1 1-e 0+e 0+e],c2);patch([0 0 1 1-e 0+e 0+e],[0 1 1 1-e 1-e 0+e],c3);plot([0 1 1 0 0],[0 0 1 1 0]);disp('weights');
  "IW{2,1}(418,:)'" : Constant  Value=[1.4591973239168272158394756843335926532745361328125;-0.45033311568191980445163835611310787498950958251953125;0.243930243676670988062227252157754264771938323974609375;0.72384725753444201234998445215751416981220245361328125;-2.37041351429839242115349406958557665348052978515625;-0.1600750338368608638450751868731458671391010284423828125;-0.8366146174533664048311720762285403907299041748046875;1.4021664418885240177559126095729880034923553466796875]
      mask Display: e = 0.06;c1 = [120 150 230]/255;c2 = ([120 150 230]+0)/383;c3 = ([120 150 230]+128)/383;patch([0 1 1 0],[0 0 1 1],c1);patch([0 1 1 1-e 1-e 0+e],[0 0 1 1-e 0+e 0+e],c2);patch([0 0 1 1-e 0+e 0+e],[0 1 1 1-e 1-e 0+e],c3);plot([0 1 1 0 0],[0 0 1 1 0]);disp('weights');
  "IW{2,1}(419,:)'" : Constant  Value=[1.1419618998867056003376774242497049272060394287109375;1.372454281466145342704976428649388253688812255859375;1.274935688426646063220459836884401738643646240234375;0.0295724390392197965249376778729129000566899776458740234375;-0.188094588913903904003888101215125061571598052978515625;1.4426533523534954550626707714400254189968109130859375;1.4655503440175092766395437138271518051624298095703125;-1.423907772155761808363649834063835442066192626953125]
      mask Display: e = 0.06;c1 = [120 150 230]/255;c2 = ([120 150 230]+0)/383;c3 = ([120 150 230]+128)/383;patch([0 1 1 0],[0 0 1 1],c1);patch([0 1 1 1-e 1-e 0+e],[0 0 1 1-e 0+e 0+e],c2);patch([0 0 1 1-e 0+e 0+e],[0 1 1 1-e 1-e 0+e],c3);plot([0 1 1 0 0],[0 0 1 1 0]);disp('weights');
  "IW{2,1}(42,:)'" : Constant  Value=[-1.479551959669791028062491022865287959575653076171875;0.73892382002569301224781384007656015455722808837890625;-0.0240968561511420674425831833787015057168900966644287109375;-1.072668296033023604962863828404806554317474365234375;-0.409415311438202145222220451614703051745891571044921875;1.4998099565215008421859010923071764409542083740234375;1.501968152198852823886454643798060715198516845703125;-1.60606832914012187529806396923959255218505859375]
      mask Display: e = 0.06;c1 = [120 150 230]/255;c2 = ([120 150 230]+0)/383;c3 = ([120 150 230]+128)/383;patch([0 1 1 0],[0 0 1 1],c1);patch([0 1 1 1-e 1-e 0+e],[0 0 1 1-e 0+e 0+e],c2);patch([0 0 1 1-e 0+e 0+e],[0 1 1 1-e 1-e 0+e],c3);plot([0 1 1 0 0],[0 0 1 1 0]);disp('weights');
  "IW{2,1}(420,:)'" : Constant  Value=[1.616209240232409971582683283486403524875640869140625;1.1171758225011110265967317900503985583782196044921875;-0.607975418850734694586890327627770602703094482421875;-1.0116019415181380924906306972843594849109649658203125;1.6278137067577056473766106137190945446491241455078125;1.243604898371561517933514551259577274322509765625;-1.176714644987587377045201719738543033599853515625;-0.1258089473179569151017886952104163356125354766845703125]
      mask Display: e = 0.06;c1 = [120 150 230]/255;c2 = ([120 150 230]+0)/383;c3 = ([120 150 230]+128)/383;patch([0 1 1 0],[0 0 1 1],c1);patch([0 1 1 1-e 1-e 0+e],[0 0 1 1-e 0+e 0+e],c2);patch([0 0 1 1-e 0+e 0+e],[0 1 1 1-e 1-e 0+e],c3);plot([0 1 1 0 0],[0 0 1 1 0]);disp('weights');
  "IW{2,1}(421,:)'" : Constant  Value=[-0.891277344279810979088551903259940445423126220703125;-0.042462772395036867123518931066428194753825664520263671875;-0.8064411167562466342673133112839423120021820068359375;-1.847918228398895745812069435487501323223114013671875;-0.1876476345440316328971874781927908770740032196044921875;1.781555302072161506288239252171479165554046630859375;-1.3345051293847693951732935602194629609584808349609375;-1.07293234297775796903806622140109539031982421875]
      mask Display: e = 0.06;c1 = [120 150 230]/255;c2 = ([120 150 230]+0)/383;c3 = ([120 150 230]+128)/383;patch([0 1 1 0],[0 0 1 1],c1);patch([0 1 1 1-e 1-e 0+e],[0 0 1 1-e 0+e 0+e],c2);patch([0 0 1 1-e 0+e 0+e],[0 1 1 1-e 1-e 0+e],c3);plot([0 1 1 0 0],[0 0 1 1 0]);disp('weights');
  "IW{2,1}(422,:)'" : Constant  Value=[-1.4744461006221205590094314175075851380825042724609375;1.200284427565353251310398263740353286266326904296875;-0.4706701174905869589082385573419742286205291748046875;-1.2046465102924457379884870533715002238750457763671875;0.776413089797364452948613688931800425052642822265625;1.3391619619007906205609970129444263875484466552734375;-1.49068541064716075794649441377259790897369384765625;-1.0664795526915853418614688052912242710590362548828125]
      mask Display: e = 0.06;c1 = [120 150 230]/255;c2 = ([120 150 230]+0)/383;c3 = ([120 150 230]+128)/383;patch([0 1 1 0],[0 0 1 1],c1);patch([0 1 1 1-e 1-e 0+e],[0 0 1 1-e 0+e 0+e],c2);patch([0 0 1 1-e 0+e 0+e],[0 1 1 1-e 1-e 0+e],c3);plot([0 1 1 0 0],[0 0 1 1 0]);disp('weights');
  "IW{2,1}(423,:)'" : Constant  Value=[-1.7681034722515687196420230975490994751453399658203125;0.0270646138684207081259724958499646163545548915863037109375;1.5599120111570179414428594100172631442546844482421875;-1.1947480484737240669090851952205412089824676513671875;0.237458348547009368001425855254638008773326873779296875;-0.89881625051539348891793679285910911858081817626953125;-1.3697081777988329154283064781338907778263092041015625;-1.2049948161896122389435959121328778564929962158203125]
      mask Display: e = 0.06;c1 = [120 150 230]/255;c2 = ([120 150 230]+0)/383;c3 = ([120 150 230]+128)/383;patch([0 1 1 0],[0 0 1 1],c1);patch([0 1 1 1-e 1-e 0+e],[0 0 1 1-e 0+e 0+e],c2);patch([0 0 1 1-e 0+e 0+e],[0 1 1 1-e 1-e 0+e],c3);plot([0 1 1 0 0],[0 0 1 1 0]);disp('weights');
  "IW{2,1}(424,:)'" : Constant  Value=[-0.92457122739501518271509894475457258522510528564453125;-1.18900291365498933515709722996689379215240478515625;-1.03235433147516797447451608604751527309417724609375;1.4510436158901993675129915573052130639553070068359375;-1.12121663221337630744756097556091845035552978515625;-1.545810588413491171166924686986021697521209716796875;1.212090047073938858801511742058210074901580810546875;-0.73571366046196196020190427589113824069499969482421875]
      mask Display: e = 0.06;c1 = [120 150 230]/255;c2 = ([120 150 230]+0)/383;c3 = ([120 150 230]+128)/383;patch([0 1 1 0],[0 0 1 1],c1);patch([0 1 1 1-e 1-e 0+e],[0 0 1 1-e 0+e 0+e],c2);patch([0 0 1 1-e 0+e 0+e],[0 1 1 1-e 1-e 0+e],c3);plot([0 1 1 0 0],[0 0 1 1 0]);disp('weights');
